simulink library "DAEMOT_Lib"  (R2019b)
settings: Solver=ode45  StartTime=0.0  StopTime=10.0  FixedStep=0.1  RelTol=1e-3
undefined symbols (not defined in the file or in its folder): Controller, CP, Ctrl, Ctrl_Fcn, Elec1, f, F2, Fluid, lag1, Mission, Moody, PropellerProp, rev_comms_sink
libraries: $bdroot x200, instrumentlib x21, simulink x5, dspsigops x2
(part 2 of 13)

== system DAEMOT_Lib/Electrical ==
  Air Vehicle : Subsystem  mask{rho=1.225, g=9.81, M=85, A=2*pi*(1/3)^2, d=.625, C_D=1.5/90, C_T=.07, C_tau=.01, eta=.95, theta=3.6, v_initial=30}
      mask prompts: rho "Air Density [kg/m^3]"; g "Gravity [m/s^2]"; M "Vehicle Mass [kg]"; A "Frontal Area [m^2]"; d "Prop Diameter"; C_D "Drag Coefficient [-]"; C_T "Thrust Coefficient [-]"; C_tau "Torque Coefficient [-]"; eta "Prop Efficiency [-]"; theta "Angle of attack [degrees]"; v_initial "Initial Vehicle Speed [m/s]"
      mask init:
      | % map = load('PropellerProp','PropellerProp');
      | % Prop = eval(['map.PropellerProp.' prop]);
      | % d = Prop.d;
      settings: CopyFcn=|
      | h      = get_param(gcb,'handle');   % Get block handle
      | blk    = gcb;
      | 
      | set_param(blk, 'LinkStatus', 'inactive')
      | clear h
      | clear blk
      mask DialogControl ParameterTabVar0 Prompt: Vehicle Parameters
      mask DialogControl ParameterTabVar012 Prompt: System
      mask Display:
      | image(imread('UAV.bmp'));
      | text(0.5,0.95,['{\bf UAV}'],'TexMode','on','horizontalAlignment', 'center')
      | text(0.5,0.075,['{\bf (\tau)  (end)}'],'TexMode','on','horizontalAlignment', 'center')
      | 
      | port_label('input',1,sprintf('Mechanical \nIn'))
      | 
      | % port_label('input',2,'\theta [rad]','interpreter','tex')
  Battery : Subsystem  AncestorBlock=DAEMOT_Lib_Copy/Dyn Electrical Comp/Battery  mask{C_c=62.7, C_s=4.5, R_cond=1.94, B_cap=21.33, Ns=3, Np=2, batt=57.6 Testbed 21.33 Ah, Ts_initial=25, Tc_initial=25, SOC_initial=.75, RC_initial=[0 0]}
      mask prompts: C_c "Lumped Cell Core Heat Capacity [J/K]"; C_s "Lumped Cell Surface Heat Capacity [J/K]"; R_cond "Conduction Resistance  [K/W]"; B_cap "Battery Capacity [Ah]"; Ns "Number of Cells (Series)"; Np "Number of Cells (Parallel)"; batt "Battery Type"; Ts_initial "Initial Battery Surface Temperature [C]"; Tc_initial "Initial Battery Core Temperature [C]"; SOC_initial "Initial State of Charge"; RC_initial "Initial RC Pair Voltage"
      mask init:
      | load('BattProp.mat');
      | 
      | if strcmp(batt,'3.3V LiFePO4 2.3 Ah')
      |     cell = BattProp.LiFePO_33V;
      |     t = 1;
      | end
      | 
      | if strcmp(batt,'3.3V LiFePO4 Graph 2.3 Ah')
      |     cell = BattProp.LiFePO_33V_G;
      |     t = 2;
      | end
      | 
      | if strcmp(batt,'4.2V LiPo 5.1 Ah')
      |     cell = BattProp.LiPo_42V;
      |     t = 1;
      | end
      | 
      | if strcmp(batt,'4.2V LiPo Graph 5.1 Ah')
      |     cell = BattProp.LiPo_42V_G;
      |     t = 2;
      | end
      | 
      | if strcmp(batt,'57.6 Testbed 21.33 Ah')
      |     cell = BattProp.Testbed4Pack;
      |     t = 1;
      | end
      | 
      | if strcmp(batt,'57.6 Testbed Graph 21.33 Ah')
      |     cell = BattProp.Testbed4Pack_G;
      |     t = 2;
      | end
      | 
      | 
      | % B_cap = B_cap*Np;
      | % C_c = C_c*Np*Ns;
      | % C_s = C_s*Np*Ns;
      | % R_cond = R_cond/(Np*Ns);
      settings: CopyFcn=|
      | h      = get_param(gcb,'handle');   % Get block handle
      | blk    = gcb;
      | 
      | set_param(blk, 'LinkStatus', 'inactive')
      | clear h
      | clear blk
      mask TypeOptions batt: 3.3V LiFePO4 2.3 Ah | 3.3V LiFePO4 Graph 2.3 Ah | 4.2V LiPo 5.1 Ah | 4.2V LiPo Graph 5.1 Ah | 57.6 Testbed 21.33 Ah | 57.6 Testbed Graph 21.33 Ah
      mask DialogControl ParameterTabVar0 Prompt: Module Parameters
      mask DialogControl ParameterTabVar01 Prompt: Initial Conditions
      mask DialogControl ParameterTabVar012 Prompt: System
      mask Display:
      | image(imread('battery.bmp'))
      | N = get_param(gcb,'Np');
      | M = get_param(gcb,'Ns');
      | 
      | text(0.5,0.95,[M '{\bfS}' N '{\bfP Battery}'],'TexMode','on','horizontalAlignment', 'center')
      | text(0.5,0.075,['{\bf (V)*}'],'TexMode','on','horizontalAlignment', 'center')
      | 
      | port_label('input',1,sprintf('Electrical \nIn'))
      | 
      | port_label('output',1,sprintf('Electrical \nOut'))
      | port_label('output',2,sprintf('Cooling \nOut'))
  Bus : Subsystem  mask{R=.1, L=.0001, C=1, Num_In=2, Num_Out=2, V_initial=.5, I_initial=0}
      mask prompts: R "Resistance [Ohm]"; L "Inductance [H]"; C "Capacitance [F]"; Num_In "Number of Inputs"; Num_Out "Number of Outputs"; V_initial "Initial Voltage [V]"; I_initial "Initial Current [A]"
      mask init:
      | h      = get_param(gcb,'handle');   % Get block handle
      | blk    = gcb;
      | hblock = get(h);     % Parse out handles structure
      | 
      | %%%%%%%%%%%%%%%%%%%%%%%%%%%%%% Clear Stuff %%%%%%%%%%%%%%%%%%%%%%%%%%%%%%%%
      | %delete any previous inports and bus selectors
      | for i = str2num(hblock.Num_In)+1:hblock.Ports(1)-2
      |     delete_block([blk,'/In',num2str(i)])
      |     delete_block([blk,'/gb',num2str(i)])
      |     delete_block([blk,'/vm',num2str(i)])
      |     delete_block([blk,'/term',num2str(i)])
      |     delete_block([blk,'/Sink',num2str(i)])
      |     delete_block([blk,'/vin',num2str(i)])
      |     
      |     delete_unconnected_lines(blk)
      | end
      | 
      | for i = str2num(hblock.Num_Out)+1:hblock.Ports(2)
      |     delete_block([blk,'/Out',num2str(i)])
      |     delete_block([blk,'/if',num2str(i)])
      |     delete_block([blk,'/io',num2str(i)])
      |     delete_block([blk,'/vo',num2str(i)])
      |     delete_block([blk,'/vot',num2str(i)])
      |     delete_block([blk,'/b',num2str(i)])
      |     delete_block([blk,'/Source',num2str(i)])
      |     delete_block([blk,'/ig',num2str(i)])
      |     delete_block([blk,'/ios',num2str(i)])
      |     
      |     delete_unconnected_lines(blk)
      | end
      | %%%%%%%%%%%%%%%%%%%%%%%%%%%%% Clear Stuff %%%%%%%%%%%%%%%%%%%%%%%%%%%%%%%%
      | 
      | %%%%%%%%%%%%%%%%%%%%%%%%%%%%%% Edit Mux inputs %%%%%%%%%%%%%%%%%%%%%%%%%%%%%%%%
      | set_param([blk,'/Mux_In_1'],'Inputs',hblock.Num_In)
      | set_param([blk,'/Mux_In_2'],'Inputs',hblock.Num_Out)
      | set_param([blk,'/Demux_Out_1'],'Outputs',hblock.Num_In)
      | set_param([blk,'/Demux_Out_2'],'Outputs',hblock.Num_Out)
      | set_param([blk,'/u_Out'],'Port',num2str(Num_In+2))
      | set_param([blk,'/u_In'],'Port',num2str(Num_In+1))
      | set_param([blk,'/Bus_Sink_1'],'Inputs',num2str(str2num(hblock.Num_Out)+1))
      | 
      | %%%%%%%%%%%%%%%%%%%%%%%%%%%%%% Edit Mux inputs %%%%%%%%%%%%%%%%%%%%%%%%%%%%%%%%
      | 
      | %%%%%%%%%%%%%%%%%%%%%%%%%%%%%% Create and Place Inputs %%%%%%%%%%%%%%%%%%%%%%%%%%%%%%%%
      | % generate inports, bus selectors, and route lines to each vector concat
      | for i = hblock.Ports(1)+1-2:str2num(hblock.Num_In)
      |     
      |     % add blocks (positioning notation [x i*s+y x+l i*s+h+y] x:(horiz. pos.), y:(vert. pos.), s:(spacing), l:(horiz. length), x:(vert. height)
      |     add_block('simulink/Ports & Subsystems/In1',   [blk,'/In',num2str(i)],    'Position',[355 i*80+425 355+30 i*80+13+425]);         % adding inport
      |     add_block([blk,'/gb1'],                        [blk,'/gb',num2str(i)],   'Position',[440 i*80+410 440+5 i*80+38+410]);         % adding inport
      |     add_block('simulink/Signal Routing/Goto',      [blk,'/vm',num2str(i)],    'Position',[500 i*80+450 500+80 i*80+14+450]);         % adding inport
      |     add_block('simulink/Sinks/Terminator',          [blk,'/term',num2str(i)],    'Position',[500 i*80+415 500+20 i*80+14+415]);         % adding inport
      |     add_block('DAEMOT_Lib/Support Functions/Sink',[blk,'/Sink',num2str(i)],'Position',[200 i*30+336 200+65 i*30+28+336]);         % adding inport
      |     add_block('simulink/Signal Routing/From',       [blk,'/vin',num2str(i)],     'Position',[-400 i*20+405 -400+80 i*20+18+405]);         % adding inport
      |     
      |     % set goto and from tags
      |     set_param([blk,'/vm',num2str(i)],'GotoTag',char(horzcat('V_in',num2str(i))))
      |     set_param([blk,'/vin',num2str(i)],'GotoTag',char(horzcat('V_in',num2str(i))))
      |     
      |     % set goto and from background colors
      | %    set_param([blk,'/gm',num2str(i)],'BackgroundColor','yellow')
      | %    set_param([blk,'/gt',num2str(i)],'BackgroundColor','yellow')
      | %    %set_param([blk,'/gp',num2str(i)],'BackgroundColor','yellow')
      | %    set_param([blk,'/min',num2str(i)],'BackgroundColor','yellow')
      | %    set_param([blk,'/tin',num2str(i)],'BackgroundColor','yellow')
      | %    set_param([blk,'/pout',num2str(i)],'BackgroundColor','cyan')
      |     
      |     % add lines
      |     add_line(blk,['In',num2str(i),'/1'], ['gb',num2str(i),'/1'],'AutoRouting','on')
      |     add_line(blk,['gb',num2str(i),'/2'],  ['vm',num2str(i),'/1'],'AutoRouting','on')
      |     add_line(blk,['gb',num2str(i),'/1'],  ['term',num2str(i),'/1'],'AutoRouting','on')
      |     add_line(blk,['Demux_Out_1/',num2str(i)],  ['Sink',num2str(i),'/1'],'AutoRouting','on')
      |     add_line(blk,['vin',num2str(i),'/1'],  ['Mux_In_1/',num2str(i)],'AutoRouting','on')
      | %     
      | end
      | %%%%%%%%%%%%%%%%%%%%%%%%%%%%%% Create and Place Inputs %%%%%%%%%%%%%%%%%%%%%%%%%%%%%%%%
      | 
      | %%%%%%%%%%%%%%%%%%%%%%%%%%%%%% Create and Place Outputs %%%%%%%%%%%%%%%%%%%%%%%%%%%%%%%%
      | % generate inports, bus selectors, and route lines to each vector concat
      | for i = hblock.Ports(2)+1:str2num(hblock.Num_Out)
      |     
      |     % add blocks
      |     add_block('simulink/Ports & Subsystems/Out1',   [blk,'/Out',num2str(i)],   'Position',[875 i*80+425 875+30 i*80+13+425]);         % adding inport
      |     add_block('simulink/Signal Routing/Bus Creator',[blk,'/b',num2str(i)],     'Position',[825 i*80+410 825+5 i*80+38+410]);         % adding inport
      |     add_block('simulink/Signal Routing/From',       [blk,'/io',num2str(i)],     'Position',[710 i*80+415 710+80 i*80+14+415]);         % adding inport
      |     add_block('simulink/Signal Routing/From',       [blk,'/vo',num2str(i)],     'Position',[710 i*80+435 710+80 i*80+14+435]);         % adding inport
      |     add_block('simulink/Signal Routing/Goto',       [blk,'/vot',num2str(i)],     'Position',[1250 i*20+50 1250+80 i*20+18+50]);         % adding inport
      |     add_block('simulink/Signal Routing/From',       [blk,'/if',num2str(i)],     'Position',[935 i*20+410 935+80 i*20+18+410]);         % adding inport
      |     add_block('DAEMOT_Lib/Support Functions/Source',[blk,'/Source',num2str(i)],'Position',[1400 i*30+420 1400+65 i*30+28+420]);         % adding inport
      |     add_block('simulink/Signal Routing/Goto',       [blk,'/ig',num2str(i)],     'Position',[1550 i*30+430 1550+80 i*30+14+430]);         % adding inport
      |     add_block('simulink/Signal Routing/From',       [blk,'/ios',num2str(i)],     'Position',[1770 i*16+405 1770+80 i*16+14+405]);         % adding inport
      |     
      |     % set goto and from tags
      |     set_param([blk,'/if',num2str(i)],'GotoTag',char(horzcat('I_out',num2str(i))))
      |     set_param([blk,'/io',num2str(i)],'GotoTag',char(horzcat('I_out',num2str(i))))
      |     set_param([blk,'/vo',num2str(i)],'GotoTag',char(horzcat('V_out',num2str(i))))
      |     set_param([blk,'/vot',num2str(i)],'GotoTag',char(horzcat('V_out',num2str(i))))
      |     set_param([blk,'/ig',num2str(i)],'GotoTag',char(horzcat('I_out',num2str(i))))
      |     set_param([blk,'/ios',num2str(i)],'GotoTag',char(horzcat('I_out',num2str(i))))
      |     set_param([blk,'/b',num2str(i)],'Inputs','2')
      |     
      | %     % set goto and from background colors
      | %     set_param([blk,'/t',num2str(i)],'BackgroundColor','cyan')
      | %     set_param([blk,'/m',num2str(i)],'BackgroundColor','cyan')
      | %     set_param([blk,'/p',num2str(i)],'BackgroundColor','cyan')
      | %     set_param([blk,'/g',num2str(i)],'BackgroundColor','cyan')
      | %     set_param([blk,'/mout',num2str(i)],'BackgroundColor','cyan')
      | %     %set_param([blk,'/tout',num2str(i)],'BackgroundColor','cyan')
      |     
      |     % add lines
      |     add_line(blk,['io',num2str(i),'/1'],['b',num2str(i),'/1'],'AutoRouting','on')
      |     p = get_param([blk,'/io',num2str(i)],'PortHandles');
      |     l = get_param(p.Outport,'Line');
      |     set_param(l,'Name','current')
      |     
      |     add_line(blk,['vo',num2str(i),'/1'],['b',num2str(i),'/2'],'AutoRouting','on')
      |     p = get_param([blk,'/vo',num2str(i)],'PortHandles');
      |     l = get_param(p.Outport,'Line');
      |     set_param(l,'Name','voltage')
      |         
      |     add_line(blk,['ios',num2str(i),'/1'],['Bus_Sink_1/',num2str(i+1)],'AutoRouting','on')
      |     p = get_param([blk,'/ios',num2str(i)],'PortHandles');
      |     l = get_param(p.Outport,'Line');
      |     set_param(l,'Name',['Current',num2str(i)])
      |      
      |     add_line(blk,['b',num2str(i),'/1'],['Out',num2str(i),'/1'],'AutoRouting','on')
      |     add_line(blk,['Source',num2str(i),'/1'],['ig',num2str(i),'/1'],'AutoRouting','on')
      |     add_line(blk,['if',num2str(i),'/1'],  ['Mux_In_2/',num2str(i)],'AutoRouting','on')
      |     add_line(blk,['Demux_Out_2/',num2str(i)],['vot',num2str(i),'/1'],'AutoRouting','on')
      |     
      | 
      | 
      | end
      | %%%%%%%%%%%%%%%%%%%%%%%%%%%%%% Create and Place Outputs %%%%%%%%%%%%%%%%%%%%%%%%%%%%%%%%
      | 
      | try
      |     set_param([blk,'/Selector1'],'InputPortWidth',num2str(hblock.Num_In))
      |     
      |     selector_str = '[1 ';
      |     for i = 2:str2num(hblock.Num_In)
      |         selector_str = [selector_str,num2str(i),' '];
      |     end
      |     selector_str = [selector_str,']'];
      |     set_param([blk,'/Selector1'],'IndexParamArray',{selector_str})%num2cell(1:hblock.Num_In))
      | catch
      |     selector_str = '[1 ';
      |     for i = 2:str2num(hblock.Num_In)
      |         selector_str = [selector_str,num2str(i),' '];
      |     end
      |     selector_str = [selector_str,']'];
      |     set_param([blk,'/Selector1'],'IndexParamArray',{selector_str})%num2cell(1:hblock.Num_In))
      |     
      |     set_param([blk,'/Selector1'],'InputPortWidth',num2str(hblock.Num_In))
      | end 
      |     
      | try
      |     set_param([blk,'/Selector2'],'InputPortWidth',num2str(hblock.Num_Out))
      |     
      |     selector_str = '[1 ';
      |     for i = 2:str2num(hblock.Num_Out)
      |         selector_str = [selector_str,num2str(i),' '];
      |     end
      |     selector_str = [selector_str,']'];
      |     set_param([blk,'/Selector2'],'IndexParamArray',{selector_str})%num2cell(1:hblock.Num_Out))
      | catch
      |     selector_str = '[1 ';
      |     for i = 2:str2num(hblock.Num_Out)
      |         selector_str = [selector_str,num2str(i),' '];
      |     end
      |     selector_str = [selector_str,']'];
      |     set_param([blk,'/Selector2'],'IndexParamArray',{selector_str})%num2cell(1:hblock.Num_Out))
      |     
      |     set_param([blk,'/Selector2'],'InputPortWidth',num2str(hblock.Num_Out))
      | end 
      | 
      |     clear h blk hblock
      settings: CopyFcn=|
      | h      = get_param(gcb,'handle');   % Get block handle
      | blk    = gcb;
      | 
      | set_param(blk, 'LinkStatus', 'inactive')
      | clear h
      | clear blk
      mask DialogControl ParameterTabVar0 Prompt: Bus Parameters
      mask DialogControl ParameterTabVar01 Prompt: System
      mask Display:
      | text(0.5,0.95,['{\bf Bus}'],'TexMode','on','horizontalAlignment', 'center')
      | text(0.5,0.075,['{\bf ----(V)}'],'TexMode','on','horizontalAlignment', 'center')
      | 
      | In = get_param(gcb,'Num_In');
      | Out = get_param(gcb,'Num_Out');
      | 
      | for i = 1:str2num(In)
      |     port_label('input',i,sprintf(['Electrical \nIn ',num2str(i)]))
      | end
      | port_label('input',str2num(In)+1,'u In')
      | port_label('input',str2num(In)+2,'u Out')
      | 
      | for i = 1:str2num(Out)
      |     port_label('output',i,sprintf(['Electrical \nOut ',num2str(i)]))
      | end
  Capacitor : Subsystem  mask{C=1, V_initial=0}
      mask prompts: C "Capacitance [F]"; V_initial "Initial Ouput Voltage [V]"
      mask init:
      | % if strcmp(Gn_check,'off')
      | %     %is not ground node
      | %     Gn = 0;
      | %     %V_initial = V_initial_temp;
      | % else
      | %     %is ground node
      | %     Gn = 1;
      | %     %V_initial = 0;
      | % end
      mask DialogControl ParameterTabVar0 Prompt: Capacitor Parameters
      mask DialogControl ParameterTabVar01 Prompt: System
      mask Display:
      | image(imread('capacitor.bmp'));
      | text(0.5,0.95,['{\bf Capacitor}'],'TexMode','on','horizontalAlignment', 'center')
      | text(0.5,0.075,['{\bf (V)}'],'TexMode','on','horizontalAlignment', 'center')
      | 
      | port_label('input',1,sprintf('Electrical \nIn'))
      | %port_label('input',2,'Capacitance')
      | port_label('output',1,sprintf('Electrical \nOut'))
  Converter : Subsystem  mask{V_D=.01, R_D=.01, R_s=.01, R_L=.01, dir=<===, Cp=60, T_initial=25}
      mask prompts: V_D "Diode Voltage Difference [V]"; R_D "Diode Resistance [Ohm]"; R_s "Switch Resistance [Ohm]"; R_L "Copper Loss [Ohm]"; dir "Conversion Direction (Boost)"; Cp "Heat Capacity [J/K]"; T_initial "Initial Temperature [C]"
      mask TypeOptions dir: ===> | <===
      mask DialogControl ParameterTabVar0 Prompt: Model Parameters
      mask DialogControl ParameterTabVar01 Prompt: Cooling
      mask DialogControl ParameterTabVar012 Prompt: System
      mask Display:
      | image(imread('converter.bmp'));
      | text(0.5,0.95,['{\bf BuckBoost Converter}'],'TexMode','on','horizontalAlignment', 'center')
      | text(0.5,0.075,['{\bf ----(V)}'],'TexMode','on','horizontalAlignment', 'center')
      | dir = get_param(gcb,'dir');
      | 
      | switch dir
      |     case '===>'
      |         text(0.5,0.85,['{\bf Boost[1] ===>}'],'TexMode','on','horizontalAlignment', 'center')
      |         text(0.5,0.75,['{\bf Buck[0] <===}'],'TexMode','on','horizontalAlignment', 'center')
      |     case '<==='
      |         text(0.5,0.85,['{\bf Boost[1] <===}'],'TexMode','on','horizontalAlignment', 'center')
      |         text(0.5,0.75,['{\bf Buck[0] ===>}'],'TexMode','on','horizontalAlignment', 'center')
      | end
      | 
      | 
      | 
      | port_label('input',1,sprintf('Electrical \nIn'))
      | port_label('input',2,sprintf('Duty \nCycle'))
      | port_label('input',3,sprintf('Operating \nMode'))
      | port_label('output',1,sprintf('Electrical \nOut'))
      | port_label('output',2,sprintf('Cooling \nOut'))
  Cooling Sink : Subsystem  Commented=on  mask(Effort Sink (Torque)){M_ext=on, M=0, T_ext=on, T=0, P_ext=on, P=0}
      mask prompts: M_ext "Mass flow rate time varying?"; M "Mass flow rate (kg/s)"; T_ext "Temperature time varying?"; T "Temperature (C)"; P_ext "Pressure time varying?"; P "Pressure (kPa)"
      mask help: Used to create a effot sink.
      mask Callback M_ext:
      | en = get_param(gcb,'MaskVisibilities');
      | h      = get_param(gcb,'handle');   % Get block handle
      | blk    = gcb;
      | hblock = get(h);     % Parse out handles structure
      | 
      | switch get_param(gcb,'M_ext')
      |     case 'on'
      |         en{2} = 'off';
      |         %add_block('simulink/Ports & Subsystems/In1',   [blk,'/In1'],'Position',[130    -7   160     7]);         % adding inport
      | 
      |     case 'off'
      |         en{2} = 'on';
      |         %delete_block([blk,'/In1'])
      | 
      | end
      | set_param(gcb,'MaskVisibilities',en);
      mask Callback T_ext:
      | en = get_param(gcb,'MaskVisibilities');
      | 
      | switch get_param(gcb,'T_ext')
      |     case 'on'
      |         en{4} = 'off';
      |     case 'off'
      |         en{4} = 'on';
      | end
      | set_param(gcb,'MaskVisibilities',en);
      mask Callback P_ext:
      | en = get_param(gcb,'MaskVisibilities');
      | 
      | switch get_param(gcb,'P_ext')
      |     case 'on'
      |         en{6} = 'off';
      |     case 'off'
      |         en{6} = 'on';
      | end
      | set_param(gcb,'MaskVisibilities',en);
      mask Display:
      | text(0.5,0.95,['{\bf Flow Sink}'],'TexMode','on','horizontalAlignment', 'center')
      | text(0.5,0.1,['{(----)(end)}'],'TexMode','on','horizontalAlignment', 'center')
      | 
      | port_label('input',1,'Sink')
      | port_label('input',2,'Sink Heat Flow [kW]')
  Cooling Source : Subsystem  Commented=on  mask(Cooling Source){M_ext=on, M=0, T_ext=on, T=0, P_ext=on, P=0}
      mask prompts: M_ext "Mass flow rate time varying?"; M "Mass flow rate (kg/s)"; T_ext "Temperature time varying?"; T "Temperature (C)"; P_ext "Pressure time varying?"; P "Pressure (kPa)"
      mask help: Used to create an cooling source.
      mask Callback M_ext:
      | en = get_param(gcb,'MaskVisibilities');
      | h      = get_param(gcb,'handle');   % Get block handle
      | blk    = gcb;
      | hblock = get(h);     % Parse out handles structure
      | 
      | switch get_param(gcb,'M_ext')
      |     case 'on'
      |         en{2} = 'off';
      |         %add_block('simulink/Ports & Subsystems/In1',   [blk,'/In1'],'Position',[130    -7   160     7]);         % adding inport
      | 
      |     case 'off'
      |         en{2} = 'on';
      |         %delete_block([blk,'/In1'])
      | 
      | end
      | set_param(gcb,'MaskVisibilities',en);
      mask Callback T_ext:
      | en = get_param(gcb,'MaskVisibilities');
      | 
      | switch get_param(gcb,'T_ext')
      |     case 'on'
      |         en{4} = 'off';
      |     case 'off'
      |         en{4} = 'on';
      | end
      | set_param(gcb,'MaskVisibilities',en);
      mask Callback P_ext:
      | en = get_param(gcb,'MaskVisibilities');
      | 
      | switch get_param(gcb,'P_ext')
      |     case 'on'
      |         en{6} = 'off';
      |     case 'off'
      |         en{6} = 'on';
      | end
      | set_param(gcb,'MaskVisibilities',en);
      mask Display:
      | text(0.5,0.95,['{\bf Effort Source}'],'TexMode','on','horizontalAlignment', 'center')
      | text(0.5,0.1,['{(start)(----)}'],'TexMode','on','horizontalAlignment', 'center')
      | 
      | port_label('input',1,sprintf('Source Heat \nFlow [kW]')  )
      | 
      | port_label('output',1,'Source')
  Current Sink : Subsystem  Commented=on  mask(Flow Sink (Current)){M_ext=on, M=0, T_ext=on, T=0, P_ext=on, P=0}
      mask prompts: M_ext "Mass flow rate time varying?"; M "Mass flow rate (kg/s)"; T_ext "Temperature time varying?"; T "Temperature (C)"; P_ext "Pressure time varying?"; P "Pressure (kPa)"
      mask help: Used to create a flow sink.
      mask Callback M_ext:
      | en = get_param(gcb,'MaskVisibilities');
      | h      = get_param(gcb,'handle');   % Get block handle
      | blk    = gcb;
      | hblock = get(h);     % Parse out handles structure
      | 
      | switch get_param(gcb,'M_ext')
      |     case 'on'
      |         en{2} = 'off';
      |         %add_block('simulink/Ports & Subsystems/In1',   [blk,'/In1'],'Position',[130    -7   160     7]);         % adding inport
      | 
      |     case 'off'
      |         en{2} = 'on';
      |         %delete_block([blk,'/In1'])
      | 
      | end
      | set_param(gcb,'MaskVisibilities',en);
      mask Callback T_ext:
      | en = get_param(gcb,'MaskVisibilities');
      | 
      | switch get_param(gcb,'T_ext')
      |     case 'on'
      |         en{4} = 'off';
      |     case 'off'
      |         en{4} = 'on';
      | end
      | set_param(gcb,'MaskVisibilities',en);
      mask Callback P_ext:
      | en = get_param(gcb,'MaskVisibilities');
      | 
      | switch get_param(gcb,'P_ext')
      |     case 'on'
      |         en{6} = 'off';
      |     case 'off'
      |         en{6} = 'on';
      | end
      | set_param(gcb,'MaskVisibilities',en);
      mask Display:
      | text(0.5,0.95,['{\bf Flow Sink}'],'TexMode','on','horizontalAlignment', 'center')
      | text(0.5,0.1,['{(----) (end)}'],'TexMode','on','horizontalAlignment', 'center')
      | 
      | port_label('input',1,'Sink')
      | port_label('input',2,'Sink Current [A]')
  Current Source : Subsystem  Commented=on  mask(Current Source){M_ext=on, M=0, T_ext=on, T=0, P_ext=on, P=0}
      mask prompts: M_ext "Mass flow rate time varying?"; M "Mass flow rate (kg/s)"; T_ext "Temperature time varying?"; T "Temperature (C)"; P_ext "Pressure time varying?"; P "Pressure (kPa)"
      mask help: Used to create an flow source.
      mask Callback M_ext:
      | en = get_param(gcb,'MaskVisibilities');
      | h      = get_param(gcb,'handle');   % Get block handle
      | blk    = gcb;
      | hblock = get(h);     % Parse out handles structure
      | 
      | switch get_param(gcb,'M_ext')
      |     case 'on'
      |         en{2} = 'off';
      |         %add_block('simulink/Ports & Subsystems/In1',   [blk,'/In1'],'Position',[130    -7   160     7]);         % adding inport
      | 
      |     case 'off'
      |         en{2} = 'on';
      |         %delete_block([blk,'/In1'])
      | 
      | end
      | set_param(gcb,'MaskVisibilities',en);
      mask Callback T_ext:
      | en = get_param(gcb,'MaskVisibilities');
      | 
      | switch get_param(gcb,'T_ext')
      |     case 'on'
      |         en{4} = 'off';
      |     case 'off'
      |         en{4} = 'on';
      | end
      | set_param(gcb,'MaskVisibilities',en);
      mask Callback P_ext:
      | en = get_param(gcb,'MaskVisibilities');
      | 
      | switch get_param(gcb,'P_ext')
      |     case 'on'
      |         en{6} = 'off';
      |     case 'off'
      |         en{6} = 'on';
      | end
      | set_param(gcb,'MaskVisibilities',en);
      mask Display:
      | text(0.5,0.95,['{\bf Flow Source}'],'TexMode','on','horizontalAlignment', 'center')
      | text(0.5,0.1,['{(start) (----)}'],'TexMode','on','horizontalAlignment', 'center')
      | 
      | %port_label('input',1,'Source Current [A]')
      | port_label('input',1,sprintf('Source \nCurrent [A]'))
      | 
      | port_label('output',1,'Source')
  ESC : Subsystem  mask{esc=NoDyno}
      mask prompts: esc "ESC Background Loss Map (filename)"
      mask init:
      | map = load('EscProp','EscProp');
      | Esc = eval(['map.EscProp.' esc]);
      settings: CopyFcn=|
      | h      = get_param(gcb,'handle');   % Get block handle
      | blk    = gcb;
      | 
      | set_param(blk, 'LinkStatus', 'inactive')
      | clear h
      | clear blk
      mask TypeOptions esc: All | NoDyno
      mask DialogControl ParameterTabVar0 Prompt: Vehicle Parameters
      mask DialogControl ParameterTabVar012 Prompt: System
      mask Display:
      | image(imread('ESC.bmp'));
      | text(0.5,0.95,['{\bf ESC Background}'],'TexMode','on','horizontalAlignment', 'center')
      | text(0.5,0.85,['{\bf Loss}'],'TexMode','on','horizontalAlignment', 'center')
      | text(0.5,0.075,['{\bf ---- (end)}'],'TexMode','on','horizontalAlignment', 'center')
      | 
      | port_label('input',1,sprintf('Electrical \nIn'))
      | % port_label('input',2,sprintf('\\lambda %g\t',10))
      | % port_label('input',2,'\theta [rad]','interpreter','tex')
  Effort Sink : Subsystem  Commented=on  mask(Effort Sink (Torque)){Stype=Voltage Sink, const=on, value=0}
      mask prompts: Stype "Sink Type"; const "Constant Value?"; value "Voltage [V]"
      mask help: Used to create a effot sink.
      mask init:
      | h      = get_param(gcb,'handle');   % Get block handle
      | blk    = gcb;
      | hblock = get(h);     % Parse out handles structure
      | 
      | if const == 1;
      |     try delete_block([blk,'/In2'])
      |         delete_unconnected_lines(blk);
      |         add_block('simulink/Sources/Constant',   [blk,'/val'], 'Position', [200,218,230,232]);
      |         add_line(blk,'val/1','Sink1/1','AutoRouting','on');
      |         set_param([blk,'/val'],'Value','value');
      |     end
      |      
      | %     delete_unconnected_lines(blk)
      | else
      |     try delete_block([blk,'/val'])
      |         delete_unconnected_lines(blk);
      |         add_block('simulink/Ports & Subsystems/In1',   [blk,'/In2'], 'Position', [200,218,230,232]);
      |         add_line(blk,'In2/1','Sink1/1','AutoRouting','on');
      |     end
      | end
      | 
      | clear h blk hblock
      settings: CopyFcn=|
      | h      = get_param(gcb,'handle');   % Get block handle
      | blk    = gcb;
      | 
      | set_param(blk, 'LinkStatus', 'inactive')
      | clear h
      | clear blk
      mask TypeOptions Stype: Voltage Sink | Current Sink | Angular Speed Sink | Torque Sink | Temperature Sink | Heat Flow Sink
      mask Callback Stype:
      | mp = get_param(gcb,'MaskPrompts');
      | h      = get_param(gcb,'handle');   % Get block handle
      | blk    = gcb;
      | hblock = get(h);     % Parse out handles structure
      | 
      | switch get_param(gcb,'Stype')
      |     case 'Voltage Sink'
      |         mp{3} = 'Voltage [V]';
      |     case 'Current Sink'
      |         mp{3} = 'Current [A]';
      |     case 'Angular Speed Sink'
      |         mp{3} = 'Speed [rad/s]';
      |     case 'Torque Sink'
      |         mp{3} = 'Torque [Nm]';
      |     case 'Temperature Sink'
      |         mp{3} = 'Temperature [C]';
      |     case 'Heat Flow Sink'
      |         mp{3} = 'Heat Flow [kW]';
      | end
      | set_param(gcb,'MaskPrompts',mp);
      mask Callback const:
      | en = get_param(gcb,'MaskVisibilities');
      | h      = get_param(gcb,'handle');   % Get block handle
      | blk    = gcb;
      | hblock = get(h);     % Parse out handles structure
      | 
      | switch get_param(gcb,'const')
      |     case 'on'
      |         en{3} = 'on';
      | %         delete_block([blk,'/In1'])
      | 
      |     case 'off'
      |         en{3} = 'off';
      | %         add_block('simulink/Ports & Subsystems/In1',   [blk,'/In1'],'Position',[130    -7   160     7]);         % adding inport
      | 
      | end
      | set_param(gcb,'MaskVisibilities',en);
      | 
      | % hblock.MaskPrompts{3} = 'hello';
      mask Display:
      | text(0.45,0.90,['{\bf',get_param(gcb,'Stype'),'}'],'TexMode','on','horizontalAlignment', 'center')
      | % text(0.5,0.1,['{(T)(end)}'],'TexMode','on','horizontalAlignment', 'center')
      | 
      | type = get_param(gcb,'Stype');
      | switch type
      |         case 'Voltage Sink'
      |             nm = 'Voltage [V]';
      |             id = '(V)';
      |             un = 'V';
      |         case 'Current Sink'
      |             nm = 'Current [A]';
      |             id = '(----)';
      |             un = 'A';
      |         case 'Angular Speed Sink'
      |             nm = 'Speed [rad/s]';
      |             id = '(----)';
      |             un = 'rad/s';
      |         case 'Torque Sink'
      |             nm = 'Torque [Nm]';
      |             id = '(\tau)';
      |             un = 'Nm';
      |         case 'Temperature Sink'
      |             nm = 'Temperature [C]';
      |             id = '(T)';
      |             un = 'C';
      |         case 'Heat Flow Sink'
      |             nm = 'Heat Flow [kW]';
      |             id = '(----)';
      |             un = 'kW';
      | end
      | 
      | if strcmp(get_param(gcb,'const'),'on')
      |     text(0.75,0.500,['{\bf',get_param(gcb,'Value'),un,'}'],'TexMode','on','horizontalAlignment', 'center')
      | else
      |     port_label('input',2,sprintf(['Sink ',nm]));
      | end
      | 
      | 
      | port_label('input',1,'Sink');
      | text(0.5,0.175,['{',id,' (end)}'],'TexMode','on','horizontalAlignment', 'center');
  Effort Source : Subsystem  Commented=on  mask(Effort Source (Voltage)){Stype=Voltage Source, const=on, value=0}
      mask prompts: Stype "Source Type"; const "Constant Value?"; value "Voltage [V]"
      mask help: Used to create an effort source.
      mask init:
      | h      = get_param(gcb,'handle');   % Get block handle
      | blk    = gcb;
      | hblock = get(h);     % Parse out handles structure
      | 
      | switch Stype
      |     case 1
      |         up = 'current';
      |         dw = 'voltage';
      |     case 2
      |         dw = 'current';
      |         up = 'voltage';
      |     case 3
      |         up = 'torque';
      |         dw = 'aspeed';
      |     case 4
      |         dw = 'torque';
      |         up = 'aspeed';
      |     case 5
      |         up = 'Q_kW';
      |         dw = 'Temp';
      |     case 6
      |         dw = 'Q_kW';
      |         up = 'Temp';
      | end
      | 
      | if const == 1;
      |     try delete_block([blk,'/In1'])
      |         delete_unconnected_lines(blk);
      |         add_block('simulink/Sources/Constant',   [blk,'/val'], 'Position', [200,198,230,212]);
      |         add_line(blk,'val/1','b1/2','AutoRouting','on');
      |         set_param([blk,'/val'],'Value','value');
      | 
      |         p = get_param([blk,'/Constant'],'PortHandles');
      |         l = get_param(p.Outport,'Line');
      |         set_param(l,'Name',up);
      |         
      |         p = get_param([blk,'/val'],'PortHandles');
      |         l = get_param(p.Outport,'Line');
      |         set_param(l,'Name',dw);
      |     end
      |     p = get_param([blk,'/Constant'],'PortHandles');
      |     l = get_param(p.Outport,'Line');
      |     if strcmp(get_param(l,'name'),up)
      |     else
      |         set_param(l,'Name',up);
      |         
      |         p = get_param([blk,'/val'],'PortHandles');
      |         l = get_param(p.Outport,'Line');
      |         set_param(l,'Name',dw);
      |     end
      |      
      | %     delete_unconnected_lines(blk)
      | else
      |     try delete_block([blk,'/val'])
      |         delete_unconnected_lines(blk);
      |         add_block('simulink/Ports & Subsystems/In1',   [blk,'/In1'], 'Position', [200,198,230,212]);
      |         add_line(blk,'In1/1','b1/2','AutoRouting','on');
      |         
      |         p = get_param([blk,'/Constant'],'PortHandles');
      |         l = get_param(p.Outport,'Line');
      |         set_param(l,'Name',up);
      | 
      |         p = get_param([blk,'/In1'],'PortHandles');
      |         l = get_param(p.Outport,'Line');
      |         set_param(l,'Name',dw);
      |     end
      |     p = get_param([blk,'/Constant'],'PortHandles');
      |     l = get_param(p.Outport,'Line');
      |     if strcmp(get_param(l,'name'),up)
      |     else
      |         set_param(l,'Name',up);
      |         
      |         p = get_param([blk,'/In1'],'PortHandles');
      |         l = get_param(p.Outport,'Line');
      |         set_param(l,'Name',dw);
      |     end
      | end
      | 
      | clear h blk hblock
      settings: CopyFcn=|
      | h      = get_param(gcb,'handle');   % Get block handle
      | blk    = gcb;
      | 
      | set_param(blk, 'LinkStatus', 'inactive')
      | clear h
      | clear blk
      mask TypeOptions Stype: Voltage Source | Current Source | Angular Speed Source | Torque Source | Temperature Source | Heat Flow Source
      mask Callback Stype:
      | mp = get_param(gcb,'MaskPrompts');
      | h      = get_param(gcb,'handle');   % Get block handle
      | blk    = gcb;
      | hblock = get(h);     % Parse out handles structure
      | 
      | switch get_param(gcb,'Stype')
      |     case 'Voltage Source'
      |         mp{3} = 'Voltage [V]';
      |     case 'Current Source'
      |         mp{3} = 'Current [A]';
      |     case 'Angular Speed Source'
      |         mp{3} = 'Speed [rad/s]';
      |     case 'Torque Source'
      |         mp{3} = 'Torque [Nm]';
      |     case 'Temperature Source'
      |         mp{3} = 'Temperature [C]';
      |     case 'Heat Flow Source'
      |         mp{3} = 'Heat Flow [kW]';
      | end
      | set_param(gcb,'MaskPrompts',mp);
      mask Callback const:
      | en = get_param(gcb,'MaskVisibilities');
      | h      = get_param(gcb,'handle');   % Get block handle
      | blk    = gcb;
      | hblock = get(h);     % Parse out handles structure
      | 
      | switch get_param(gcb,'const')
      |     case 'on'
      |         en{3} = 'on';
      | %         delete_block([blk,'/In1'])
      | 
      |     case 'off'
      |         en{3} = 'off';
      | %         add_block('simulink/Ports & Subsystems/In1',   [blk,'/In1'],'Position',[130    -7   160     7]);         % adding inport
      | 
      | end
      | set_param(gcb,'MaskVisibilities',en);
      | 
      | % hblock.MaskPrompts{3} = 'hello';
      mask Display:
      | text(0.45,0.900,['{\bf',get_param(gcb,'Stype'),'}'],'TexMode','on','horizontalAlignment', 'center')
      | 
      | type = get_param(gcb,'Stype');
      | switch type
      |         case 'Voltage Source'
      |             nm = 'Voltage [V]';
      |             id = '(V)*';
      |             un = 'V';
      |         case 'Current Source'
      |             nm = 'Current [A]';
      |             id = '(----)';
      |             un = 'A';
      |         case 'Angular Speed Source'
      |             nm = 'Speed [rad/s]';
      |             id = '(----)';
      |             un = 'rad/s';
      |         case 'Torque Source'
      |             nm = 'Torque [Nm]';
      |             id = '(\tau)*';
      |             un = 'Nm';
      |         case 'Temperature Source'
      |             nm = 'Temperature [C]';
      |             id = '(T)';
      |             un = 'C';
      |         case 'Heat Flow Source'
      |             nm = 'Heat Flow [kW]';
      |             id = '(----)';
      |             un = 'kW';
      | end
      | 
      | if strcmp(get_param(gcb,'const'),'on')
      |     text(0.25,0.500,['{\bf',get_param(gcb,'Value'),un,'}'],'TexMode','on','horizontalAlignment', 'center')
      | else
      |     port_label('input',1,sprintf(['Source \n',nm]))
      | end
      | port_label('output',1,'Source')
      | text(0.5,0.175,['{(start) ',id,'}'],'TexMode','on','horizontalAlignment', 'center')
  Engine : Subsystem  mask{G=-1, I_coeffs=[0,63.288903716034200,0], B_coeffs=[-0.015150028280914,1.757501363754273], S_coeffs=[0.197172947336021,0.088505107520121,1.502179108800752e+03,0.246955231644008,-31.725066916739816,-20.969196076216960], tau=.5, I_initial=0}
      mask prompts: G "Current Gain"; I_coeffs "Current Coefficients"; B_coeffs "Current Bound Coefficients"; S_coeffs "SFC Coefficients"; tau "Time Constant [s]"; I_initial "Initial Current"
      mask init:
      | % SFC_max = max(2);
      | % u_min = min(1);
      | % SFC_min = min(2);
      | % 
      | % a = -(SFC_min-SFC_max)/(u_min^2);
      | % b = -2*a*u_min;
      | % c = SFC_max;
      | 
      | S = [S_coeffs(1)   S_coeffs(4)/2 S_coeffs(5)/2; ...
      |      S_coeffs(4)/2 S_coeffs(2)   S_coeffs(6)/2; ...
      |      S_coeffs(5)/2 S_coeffs(6)/2 S_coeffs(3)];
      mask DialogControl ParameterTabVar0 Prompt: Engine Parameters
      mask DialogControl ParameterTabVar012 Prompt: System
      mask Display:
      | image(imread('generator.bmp'));
      | text(0.5,0.95,['{\bf Engine}'],'TexMode','on','horizontalAlignment', 'center')
      | text(0.5,0.075,['{\bf (----) (end)}'],'TexMode','on','horizontalAlignment', 'center')
      | 
      | port_label('input',1,sprintf('Electrical \nIn'))
      | port_label('input',2,sprintf('Throttle \n[%%]'))
  Gearbox : Subsystem  Commented=on  AncestorBlock=DAEMOT_Lib_Copy/Dyn Electrical Comp/Gearbox  mask{R=5, dir=1}
      mask prompts: R "Gear Ratio"; dir "Type"
      mask init:
      | h      = get_param(gcb,'handle');   % Get block handle
      | blk    = gcb;
      | hblock = get(h);     % Parse out handles structure
      | 
      | 
      | if dir == 1
      |     set_param([blk,'/i1'],'GotoTag',char(horzcat('term')));
      |     set_param([blk,'/i2'],'GotoTag',char(horzcat('var_in')));
      |     set_param([blk,'/O1'],'GotoTag',char(horzcat('in_down')));
      |     set_param([blk,'/O2'],'GotoTag',char(horzcat('var_out')));
      |     
      |     set_param([blk,'/o1'],'GotoTag',char(horzcat('out_up')));
      |     p = get_param([blk,'/o1'],'PortHandles');
      |     l = get_param(p.Outport,'Line');
      |     set_param(l,'Name','Input Speed [rad_s]')
      |     
      |     set_param([blk,'/o2'],'GotoTag',char(horzcat('var_out')));
      |     p = get_param([blk,'/o2'],'PortHandles');
      |     l = get_param(p.Outport,'Line');
      |     set_param(l,'Name','Output Torque [Nm]')
      | else
      |     set_param([blk,'/i1'],'GotoTag',char(horzcat('var_in')));
      |     set_param([blk,'/i2'],'GotoTag',char(horzcat('term')));
      |     set_param([blk,'/O1'],'GotoTag',char(horzcat('var_out')));
      |     set_param([blk,'/O2'],'GotoTag',char(horzcat('in_down')));
      |     
      |     set_param([blk,'/o1'],'GotoTag',char(horzcat('var_out')));
      |     p = get_param([blk,'/o1'],'PortHandles');
      |     l = get_param(p.Outport,'Line');
      |     set_param(l,'Name','Output Speed [rad_s]')
      |     
      |     set_param([blk,'/o2'],'GotoTag',char(horzcat('out_up')));
      |     p = get_param([blk,'/o2'],'PortHandles');
      |     l = get_param(p.Outport,'Line');
      |     set_param(l,'Name','Input Torque [Nm]')
      | end
      settings: CopyFcn=|
      | h      = get_param(gcb,'handle');   % Get block handle
      | blk    = gcb;
      | 
      | set_param(blk, 'LinkStatus', 'inactive')
      | clear h
      | clear blk
      mask TypeOptions dir: 1 | 2
      mask DialogControl ParameterTabVar0 Prompt: Gearbox Parameters
      mask DialogControl ParameterTabVar012 Prompt: System
      mask Display:
      | image(imread('Gearbox.bmp'));
      | text(0.5,0.95,['{\bf Gearbox}'],'TexMode','on','horizontalAlignment', 'center')
      | dir = get_param(gcb,'dir');
      | 
      | switch dir
      |     case '1'
      |         text(0.5,0.075,['{\bf ----(\tau)}'],'TexMode','on','horizontalAlignment', 'center')
      |     case '2'
      |         text(0.5,0.075,['{\bf (\tau)----}'],'TexMode','on','horizontalAlignment', 'center')
      | end
      | 
      | 
      | 
      | port_label('input',1,sprintf('Mech. \nIn'))
      | port_label('output',1,sprintf('Mech. \nOut'))
  Generator : Subsystem  Commented=on  mask{G=2.25}
      mask prompts: G "Current Gain"
      mask init:
      | load('Eng3W.mat')
      | 
      | cI = Eng3W.cI;
      | cSFC = Eng3W.cSFC;
      | mu_V = Eng3W.mu_V;
      | std_V = Eng3W.std_V;
      | mu_u = Eng3W.mu_u;
      | std_u = Eng3W.std_u;
      mask DialogControl ParameterTabVar0 Prompt: Generator Parameters
      mask DialogControl ParameterTabVar012 Prompt: System
      mask Display:
      | image(imread('generator.bmp'));
      | text(0.5,0.95,['{\bf Generator}'],'TexMode','on','horizontalAlignment', 'center')
      | text(0.5,0.075,['{\bf (--)}'],'TexMode','on','horizontalAlignment', 'center')
      | 
      | port_label('input',1,sprintf('Electrical \nIn'))
      | port_label('input',2,sprintf('Throttle \n[%%]'))
  Ground Vehicle : Subsystem  mask{R=.3, Af=2, rho_air=1.2, Cd=.26}
      mask prompts: R "Wheel Radius [m]"; Af "Frontal Area [m^2]"; rho_air "Air Density [kg/m^3]"; Cd "Drag Coefficient [-]"
      mask init:
      | % if strcmp(Gn_check,'off')
      | %     %is not ground node
      | %     Gn = 0;
      | %     %V_initial = V_initial_temp;
      | % else
      | %     %is ground node
      | %     Gn = 1;
      | %     %V_initial = 0;
      | % end
      mask DialogControl ParameterTabVar0 Prompt: Capacitor Parameters
      mask DialogControl ParameterTabVar01 Prompt: System
      mask Display:
      | image(imread('ground.bmp'));
      | text(0.5,0.95,['{\bf Ground Vehicle}'],'TexMode','on','horizontalAlignment', 'center')
      | text(0.5,0.075,['{\bf (T)  (end)}'],'TexMode','on','horizontalAlignment', 'center')
      | 
      | port_label('input',1,sprintf('Mechanical \nIn'))
      | port_label('input',2,sprintf('Brake \nTorque [Nm]'))
  Inductor : Subsystem  mask{L=1, I_initial=0}
      mask prompts: L "Inductance [H]"; I_initial "Initial Current [A]"
      mask init:
      | % if strcmp(Gn_check,'off')
      | %     %is not ground node
      | %     Gn = 0;
      | %     %V_initial = V_initial_temp;
      | % else
      | %     %is ground node
      | %     Gn = 1;
      | %     %V_initial = 0;
      | % end
      mask DialogControl ParameterTabVar0 Prompt: Capacitor Parameters
      mask DialogControl ParameterTabVar01 Prompt: System
      mask Display:
      | image(imread('inductor.bmp'));
      | text(0.5,0.95,['{\bf Inductor}'],'TexMode','on','horizontalAlignment', 'center')
      | text(0.5,0.075,['{\bf ----}'],'TexMode','on','horizontalAlignment', 'center')
      | 
      | port_label('input',1,sprintf('Electrical \nIn'))
      | %port_label('input',2,'Inductance')
      | port_label('output',1,sprintf('Electrical \nOut'))
  Inverter : Subsystem  mask{R_m=.0808, Cp=10000, T_initial=25}
      mask prompts: R_m "Modulated Loss [Ohm]"; Cp "Heat Capacity [J/K]"; T_initial "Initial Temperature [C]"
      settings: CopyFcn=|
      | h      = get_param(gcb,'handle');   % Get block handle
      | blk    = gcb;
      | 
      | set_param(blk, 'LinkStatus', 'inactive')
      | clear h
      | clear blk
      mask DialogControl DescTextVar Prompt: This is a wye configured inverter.
      mask DialogControl ParameterTabVar0 Prompt: Inverter Parameters
      mask DialogControl ParameterTabVar01 Prompt: Cooling
      mask DialogControl ParameterTabVar012 Prompt: System
      mask Display:
      | image(imread('inverter.bmp'));
      | text(0.5,0.95,['{\bf Inverter}'],'TexMode','on','horizontalAlignment', 'center')
      | text(0.5,0.075,['{\bf ----(V)}'],'TexMode','on','horizontalAlignment', 'center')
      | 
      | 
      | % switch dir
      | %     case '===>'
      | %         text(0.5,0.85,['{\bf Boost[1] ===>}'],'TexMode','on','horizontalAlignment', 'center')
      | %         text(0.5,0.75,['{\bf Buck[0] <===}'],'TexMode','on','horizontalAlignment', 'center')
      | %     case '<==='
      | %         text(0.5,0.85,['{\bf Boost[1] <===}'],'TexMode','on','horizontalAlignment', 'center')
      | %         text(0.5,0.75,['{\bf Buck[0] ===>}'],'TexMode','on','horizontalAlignment', 'center')
      | % end
      | 
      | 
      | 
      | port_label('input',1,sprintf('Electrical \nIn'))
      | port_label('input',2,sprintf('Modulation'))
      | % port_label('input',3,'Operating Mode')
      | port_label('output',1,sprintf('Electrical \nOut'))
      | port_label('output',2,sprintf('Cooling \nOut'))
  Inverter_v1 : Subsystem  Commented=on  mask{R1=.01, R2=.01, R3=.01, Cp=60, T_initial=25}
      mask prompts: R1 "Input Voltage Loss Resistance [Ohm]"; R2 "Input Current Loss Resistance [Ohm]"; R3 "Output Voltage Loss Resistance [Ohm]"; Cp "Heat Capacity [J/K]"; T_initial "Initial Temperature [C]"
      mask DialogControl ParameterTabVar0 Prompt: Model Parameters
      mask DialogControl ParameterTabVar01 Prompt: Cooling
      mask DialogControl ParameterTabVar012 Prompt: System
      mask Display:
      | image(imread('inverter.bmp'));
      | text(0.5,0.95,['{\bf Inverter}'],'TexMode','on','horizontalAlignment', 'center')
      | text(0.5,0.075,['{\bf ----(V)}'],'TexMode','on','horizontalAlignment', 'center')
      | 
      | 
      | % switch dir
      | %     case '===>'
      | %         text(0.5,0.85,['{\bf Boost[1] ===>}'],'TexMode','on','horizontalAlignment', 'center')
      | %         text(0.5,0.75,['{\bf Buck[0] <===}'],'TexMode','on','horizontalAlignment', 'center')
      | %     case '<==='
      | %         text(0.5,0.85,['{\bf Boost[1] <===}'],'TexMode','on','horizontalAlignment', 'center')
      | %         text(0.5,0.75,['{\bf Buck[0] ===>}'],'TexMode','on','horizontalAlignment', 'center')
      | % end
      | 
      | 
      | 
      | port_label('input',1,sprintf('Electrical \nIn'))
      | port_label('input',2,sprintf('Duty \nCycle'))
      | % port_label('input',3,'Operating Mode')
      | port_label('output',1,sprintf('Electrical \nOut'))
      | port_label('output',2,sprintf('Cooling \nOut'))
  Motor : Subsystem  AncestorBlock=DAEMOT_Lib_Copy/Dyn Electrical Comp/Motor  mask{m_type=AC, R=0.013461960749493, Kv=0.009688163543703, c=0.000234355495215172, b=1.89435163576232e-05, L=1.252192537082724e-05, J=1.09*10^-4, I_initial=1, w_initial=1, Cp=60, T_initial=25}
      mask prompts: m_type "Motor Type"; R "Armature Resistance [Ohm]"; Kv "Motor Constant [Nm/A] or [V-s/rad]"; c "Static Friction Coefficient [Nm]"; b "Viscous Friction Coefficient [N*m*s/rad]"; L "Armature Inductance [H]"; J "Shaft Inertia [kg*m^2]"; I_initial "Initial Total Current [A]"; w_initial "Initial Speed [rad/s]"; Cp "Motor Heat Capacity [J/K]"; T_initial "Initial Temperature [C]"
      settings: CopyFcn=|
      | h      = get_param(gcb,'handle');   % Get block handle
      | blk    = gcb;
      | 
      | set_param(blk, 'LinkStatus', 'inactive')
      | clear h
      | clear blk
      mask TypeOptions m_type: DC | AC
      mask DialogControl ParameterTabVar0 Prompt: Motor Parameters
      mask DialogControl ParameterTabVar01 Prompt: Cooling
      mask DialogControl ParameterTabVar012 Prompt: System
      mask Display:
      | image(imread('motor.bmp'));
      | T = get_param(gcb,'m_type');
      | if strcmp(T,'DC')
      |     text(0.5,0.95,['{\bf DC Motor}'],'TexMode','on','horizontalAlignment', 'center')
      | else
      |     text(0.5,0.95,['{\bf AC Motor}'],'TexMode','on','horizontalAlignment', 'center')
      | end
      | text(0.5,0.075,['{\bf ---- (end)}'],'TexMode','on','horizontalAlignment', 'center')
      | text(0.5,0.175,['{\bf (start) ----}'],'TexMode','on','horizontalAlignment', 'center')
      | 
      | port_label('input',1,sprintf('Electrical \nIn'))
      | port_label('output',1,sprintf('Mechanical \nOut'))
      | port_label('output',2,sprintf('Cooling \nOut'))
  MotorNoShaft : Subsystem  Commented=on  AncestorBlock=DAEMOT_Lib_Copy/Dyn Electrical Comp/MotorNoShaft  mask{m_type=AC, R=29e-3, Kv=.1238, c=.001, b=1e-5, L=49e-6, I_initial=1, Cp=60, T_initial=25}
      mask prompts: m_type "Motor Type"; R "Armature Resistance [Ohm]"; Kv "Motor Constant [Nm/A] or [V-s/rad]"; c "Static Friction Coefficient [Nm]"; b "Viscous Friction Coefficient [N*m*s/rad]"; L "Armature Inductance [H]"; I_initial "Initial Total Current [A]"; Cp "Motor Heat Capacity [J/K]"; T_initial "Initial Temperature [C]"
      settings: CopyFcn=|
      | h      = get_param(gcb,'handle');   % Get block handle
      | blk    = gcb;
      | 
      | set_param(blk, 'LinkStatus', 'inactive')
      | clear h
      | clear blk
      mask TypeOptions m_type: DC | AC
      mask DialogControl DescTextVar Prompt: For AC machines, parameters are defined using the Power-Invariant Park Transform.
      mask DialogControl ParameterTabVar0 Prompt: Motor Parameters
      mask DialogControl ParameterTabVar01 Prompt: Cooling
      mask DialogControl ParameterTabVar012 Prompt: System
      mask Display:
      | image(imread('motor.bmp'));
      | T = get_param(gcb,'m_type');
      | if strcmp(T,'DC')
      |     text(0.5,0.95,['{\bf DC Motor}'],'TexMode','on','horizontalAlignment', 'center')
      | else
      |     text(0.5,0.95,['{\bf AC Motor}'],'TexMode','on','horizontalAlignment', 'center')
      | end
      | text(0.5,0.075,['{\bf ---- (end)}'],'TexMode','on','horizontalAlignment', 'center')
      | text(0.5,0.175,['{\bf (start) (\tau)}'],'TexMode','on','horizontalAlignment', 'center')
      | 
      | port_label('input',1,sprintf('Electrical \nIn'))
      | port_label('output',1,sprintf('Mechanical \nOut'))
      | port_label('output',2,sprintf('Cooling \nOut'))
  Resistor : Subsystem  mask{r_type=Current, Cp=60, T_initial=25}
      mask prompts: r_type "Resistor Type"; Cp "Heat Capacity [J/K]"; T_initial "Initial Temperature [C]"
      mask init:
      | h      = get_param(gcb,'handle');   % Get block handle
      | blk    = gcb;
      | hblock = get(h);     % Parse out handles structure
      | 
      | if r_type == 1
      |     set_param([blk,'/From8'],'GotoTag',char('out'));
      |     set_param([blk,'/From10'],'GotoTag',char('in'));
      |     set_param([blk,'/From12'],'GotoTag',char('out'));
      |     set_param([blk,'/From4'],'GotoTag',char('out'));
      |     set_param([blk,'/From3'],'GotoTag',char('in'));
      | else
      |     set_param([blk,'/From8'],'GotoTag',char('in'));
      |     set_param([blk,'/From10'],'GotoTag',char('out'));
      |     set_param([blk,'/From12'],'GotoTag',char('in'));
      |     set_param([blk,'/From4'],'GotoTag',char('in'));
      |     set_param([blk,'/From3'],'GotoTag',char('out'));
      | end
      settings: CopyFcn=|
      | h      = get_param(gcb,'handle');   % Get block handle
      | blk    = gcb;
      | 
      | set_param(blk, 'LinkStatus', 'inactive')
      | clear h
      | clear blk
      mask TypeOptions r_type: Voltage | Current
      mask DialogControl ParameterTabVar0 Prompt: Resistor Parameters
      mask DialogControl ParameterTabVar01 Prompt: Cooling
      mask DialogControl ParameterTabVar012 Prompt: System
      mask Display:
      | image(imread('resistor.bmp'));
      | T = get_param(gcb,'r_type');
      | text(0.5,0.95,['{\bf Resistor}'],'TexMode','on','horizontalAlignment', 'center')
      | if strcmp(T,'Current')
      |     text(0.5,0.075,['{\bf (V)*}'],'TexMode','on','horizontalAlignment', 'center')
      | else
      |     text(0.5,0.075,['{\bf ----}'],'TexMode','on','horizontalAlignment', 'center')
      | end
      | port_label('input',1,sprintf('Electrical \nIn'))
      | port_label('input',2,sprintf('Resistance \n[Ohm]'))
      | port_label('output',1,sprintf('Electrical \nOut'))
      | port_label('output',2,sprintf('Cooling \nOut'))
  Shaft : Subsystem  Commented=on  AncestorBlock=DAEMOT_Lib_Copy/Dyn Electrical Comp/Shaft  mask{J=1.09*10^-4, Num_In=1, Num_Out=1, w_initial=0, meme=off}
      mask prompts: J "Shaft Inertia"; Num_In "Number of Inputs"; Num_Out "Number of Outputs"; w_initial "Initial Speed [rad/s]"; meme "Memify"
      mask init:
      | h      = get_param(gcb,'handle');   % Get block handle
      | blk    = gcb;
      | hblock = get(h);     % Parse out handles structure
      | 
      | %%%%%%%%%%%%%%%%%%%%%%%%%%%%%% Clear Stuff %%%%%%%%%%%%%%%%%%%%%%%%%%%%%%%%
      | %delete any previous inports and bus selectors
      | for i = str2num(hblock.Num_In)+1:hblock.Ports(1)
      |     delete_block([blk,'/In',num2str(i)])
      |     delete_block([blk,'/gb',num2str(i)])
      |     delete_block([blk,'/tm',num2str(i)])
      |     delete_block([blk,'/term',num2str(i)])
      |     delete_block([blk,'/Sink',num2str(i)])
      |     delete_block([blk,'/tin',num2str(i)])
      |     
      |     delete_unconnected_lines(blk)
      | end
      | 
      | for i = str2num(hblock.Num_Out)+1:hblock.Ports(2)
      |     delete_block([blk,'/Out',num2str(i)])
      |     delete_block([blk,'/tf',num2str(i)])
      |     delete_block([blk,'/to',num2str(i)])
      |     delete_block([blk,'/b',num2str(i)])
      |     delete_block([blk,'/Source',num2str(i)])
      |     delete_block([blk,'/tg',num2str(i)])
      |     delete_block([blk,'/oo',num2str(i)])
      |     
      |     delete_unconnected_lines(blk)
      | end
      | %%%%%%%%%%%%%%%%%%%%%%%%%%%%% Clear Stuff %%%%%%%%%%%%%%%%%%%%%%%%%%%%%%%%
      | 
      | %%%%%%%%%%%%%%%%%%%%%%%%%%%%%% Edit Mux inputs %%%%%%%%%%%%%%%%%%%%%%%%%%%%%%%%
      | set_param([blk,'/Mux_In_1'],'Inputs',hblock.Num_In)
      | set_param([blk,'/Mux_In_2'],'Inputs',hblock.Num_Out)
      | % set_param([blk,'/Demux_Out_1'],'Outputs',hblock.Num_In)
      | delete_unconnected_lines(blk)
      | 
      | %%%%%%%%%%%%%%%%%%%%%%%%%%%%%% Edit Mux inputs %%%%%%%%%%%%%%%%%%%%%%%%%%%%%%%%
      | 
      | %%%%%%%%%%%%%%%%%%%%%%%%%%%%%% Create and Place Inputs %%%%%%%%%%%%%%%%%%%%%%%%%%%%%%%%
      | % generate inports, bus selectors, and route lines to each vector concat
      | for i = hblock.Ports(1)+1:str2num(hblock.Num_In)
      |     
      |     % add blocks (positioning notation [x i*s+y x+l i*s+h+y] x:(horiz. pos.), y:(vert. pos.), s:(spacing), l:(horiz. length), x:(vert. height)
      |     add_block('simulink/Ports & Subsystems/In1',   [blk,'/In',num2str(i)],    'Position',[355 i*80+425 355+30 i*80+13+425]);         % adding inport
      |     add_block([blk,'/gb1'],                        [blk,'/gb',num2str(i)],   'Position',[440 i*80+410 440+5 i*80+38+410]);         % adding inport
      |     add_block('simulink/Signal Routing/Goto',      [blk,'/tm',num2str(i)],    'Position',[500 i*80+450 500+80 i*80+14+450]);         % adding inport
      |     add_block('simulink/Sinks/Terminator',          [blk,'/term',num2str(i)],    'Position',[500 i*80+415 500+20 i*80+14+415]);         % adding inport
      |     add_block('DAEMOT_Lib/Support Functions/Sink',[blk,'/Sink',num2str(i)],'Position',[200 i*30+336 200+65 i*30+28+336]);         % adding inport
      |     add_block('simulink/Signal Routing/From',       [blk,'/tin',num2str(i)],     'Position',[-400 i*20+405 -400+80 i*20+18+405]);         % adding inport
      |     
      |     % set goto and from tags
      |     set_param([blk,'/tm',num2str(i)],'GotoTag',char(horzcat('tau_in',num2str(i))))
      |     set_param([blk,'/tin',num2str(i)],'GotoTag',char(horzcat('tau_in',num2str(i))))
      |     
      |     % set goto and from background colors
      | %    set_param([blk,'/gm',num2str(i)],'BackgroundColor','yellow')
      | %    set_param([blk,'/gt',num2str(i)],'BackgroundColor','yellow')
      | %    %set_param([blk,'/gp',num2str(i)],'BackgroundColor','yellow')
      | %    set_param([blk,'/min',num2str(i)],'BackgroundColor','yellow')
      | %    set_param([blk,'/tin',num2str(i)],'BackgroundColor','yellow')
      | %    set_param([blk,'/pout',num2str(i)],'BackgroundColor','cyan')
      |     
      |     % add lines
      |     add_line(blk,['In',num2str(i),'/1'], ['gb',num2str(i),'/1'],'AutoRouting','on')
      |     add_line(blk,['gb',num2str(i),'/2'],  ['tm',num2str(i),'/1'],'AutoRouting','on')
      |     add_line(blk,['gb',num2str(i),'/1'],  ['term',num2str(i),'/1'],'AutoRouting','on')
      |     add_line(blk,['Demux_Out_1/',num2str(1)],  ['Sink',num2str(i),'/1'],'AutoRouting','on')
      |     add_line(blk,['tin',num2str(i),'/1'],  ['Mux_In_1/',num2str(i)],'AutoRouting','on')
      |     
      | end
      | %%%%%%%%%%%%%%%%%%%%%%%%%%%%%% Create and Place Inputs %%%%%%%%%%%%%%%%%%%%%%%%%%%%%%%%
      | 
      | %%%%%%%%%%%%%%%%%%%%%%%%%%%%%% Create and Place Outputs %%%%%%%%%%%%%%%%%%%%%%%%%%%%%%%%
      | % generate inports, bus selectors, and route lines to each vector concat
      | for i = hblock.Ports(2)+1:str2num(hblock.Num_Out)
      |     
      |     % add blocks
      |     add_block('simulink/Ports & Subsystems/Out1',   [blk,'/Out',num2str(i)],   'Position',[875 i*80+425 875+30 i*80+13+425]);         % adding inport
      |     add_block('simulink/Signal Routing/Bus Creator',[blk,'/b',num2str(i)],     'Position',[825 i*80+410 825+5 i*80+38+410]);         % adding inport
      |     add_block('simulink/Signal Routing/From',       [blk,'/to',num2str(i)],     'Position',[710 i*80+435 710+80 i*80+14+435]);         % adding inport
      |     add_block('simulink/Signal Routing/From',       [blk,'/oo',num2str(i)],     'Position',[710 i*80+415 710+80 i*80+14+415]);         % adding inport
      |     add_block('simulink/Signal Routing/From',       [blk,'/tf',num2str(i)],     'Position',[935 i*20+410 935+80 i*20+18+410]);         % adding inport
      |     add_block('DAEMOT_Lib/Support Functions/Source',[blk,'/Source',num2str(i)],'Position',[1400 i*30+420 1400+65 i*30+28+420]);         % adding inport
      |     add_block('simulink/Signal Routing/Goto',       [blk,'/tg',num2str(i)],     'Position',[1550 i*30+430 1550+80 i*30+14+430]);         % adding inport
      |     
      |     % set goto and from tags
      |     set_param([blk,'/tf',num2str(i)],'GotoTag',char(horzcat('tau_out',num2str(i))))
      |     set_param([blk,'/to',num2str(i)],'GotoTag',char(horzcat('tau_out',num2str(i))))
      |     set_param([blk,'/oo',num2str(i)],'GotoTag',char(horzcat('omega')))
      |     set_param([blk,'/tg',num2str(i)],'GotoTag',char(horzcat('tau_out',num2str(i))))
      |     set_param([blk,'/b',num2str(i)],'Inputs','2')
      |     
      | %     % set goto and from background colors
      | %     set_param([blk,'/t',num2str(i)],'BackgroundColor','cyan')
      | %     set_param([blk,'/m',num2str(i)],'BackgroundColor','cyan')
      | %     set_param([blk,'/p',num2str(i)],'BackgroundColor','cyan')
      | %     set_param([blk,'/g',num2str(i)],'BackgroundColor','cyan')
      | %     set_param([blk,'/mout',num2str(i)],'BackgroundColor','cyan')
      | %     %set_param([blk,'/tout',num2str(i)],'BackgroundColor','cyan')
      | 
      |     add_line(blk,['oo',num2str(i),'/1'],['b',num2str(i),'/1'],'AutoRouting','on')
      |     p = get_param([blk,'/oo',num2str(i)],'PortHandles');
      |     l = get_param(p.Outport,'Line');
      |     set_param(l,'Name','aspeed')
      |     
      |     add_line(blk,['to',num2str(i),'/1'],['b',num2str(i),'/2'],'AutoRouting','on')
      |     p = get_param([blk,'/to',num2str(i)],'PortHandles');
      |     l = get_param(p.Outport,'Line');
      |     set_param(l,'Name','torque')
      |      
      |     add_line(blk,['b',num2str(i),'/1'],['Out',num2str(i),'/1'],'AutoRouting','on')
      |     add_line(blk,['Source',num2str(i),'/1'],['tg',num2str(i),'/1'],'AutoRouting','on')
      |     add_line(blk,['tf',num2str(i),'/1'],  ['Mux_In_2/',num2str(i)],'AutoRouting','on')
      |     
      | 
      | 
      | end
      | %%%%%%%%%%%%%%%%%%%%%%%%%%%%%% Create and Place Outputs %%%%%%%%%%%%%%%%%%%%%%%%%%%%%%%%
      | 
      | try
      |     set_param([blk,'/Selector1'],'InputPortWidth',num2str(hblock.Num_In))
      |     
      |     selector_str = '[1 ';
      |     for i = 2:str2num(hblock.Num_In)
      |         selector_str = [selector_str,num2str(i),' '];
      |     end
      |     selector_str = [selector_str,']'];
      |     set_param([blk,'/Selector1'],'IndexParamArray',{selector_str})%num2cell(1:hblock.Num_In))
      | catch
      |     selector_str = '[1 ';
      |     for i = 2:str2num(hblock.Num_In)
      |         selector_str = [selector_str,num2str(i),' '];
      |     end
      |     selector_str = [selector_str,']'];
      |     set_param([blk,'/Selector1'],'IndexParamArray',{selector_str})%num2cell(1:hblock.Num_In))
      |     
      |     set_param([blk,'/Selector1'],'InputPortWidth',num2str(hblock.Num_In))
      | end 
      |     
      | try
      |     set_param([blk,'/Selector2'],'InputPortWidth',num2str(hblock.Num_Out))
      |     
      |     selector_str = '[1 ';
      |     for i = 2:str2num(hblock.Num_Out)
      |         selector_str = [selector_str,num2str(i),' '];
      |     end
      |     selector_str = [selector_str,']'];
      |     set_param([blk,'/Selector2'],'IndexParamArray',{selector_str})%num2cell(1:hblock.Num_Out))
      | catch
      |     selector_str = '[1 ';
      |     for i = 2:str2num(hblock.Num_Out)
      |         selector_str = [selector_str,num2str(i),' '];
      |     end
      |     selector_str = [selector_str,']'];
      |     set_param([blk,'/Selector2'],'IndexParamArray',{selector_str})%num2cell(1:hblock.Num_Out))
      |     
      |     set_param([blk,'/Selector2'],'InputPortWidth',num2str(hblock.Num_Out))
      | end 
      | 
      |     clear h blk hblock
      settings: CopyFcn=|
      | h      = get_param(gcb,'handle');   % Get block handle
      | blk    = gcb;
      | 
      | set_param(blk, 'LinkStatus', 'inactive')
      | clear h
      | clear blk
      mask DialogControl ParameterTabVar0 Prompt: Bus Parameters
      mask DialogControl ParameterTabVar01 Prompt: System
      mask Display:
      | meme = get_param(gcb,'meme');
      | if strcmp(meme,'on')
      |     image(imread('ShaftMeme.bmp'));
      | else
      |     image(imread('Shaft.bmp'));
      | end
      | text(0.5,0.95,['{\bf Shaft}'],'TexMode','on','horizontalAlignment', 'center')
      | text(0.5,0.075,['{\bf ----}'],'TexMode','on','horizontalAlignment', 'center')
      | 
      | In = get_param(gcb,'Num_In');
      | Out = get_param(gcb,'Num_Out');
      | 
      | for i = 1:str2num(In)
      |     port_label('input',i,sprintf(['Mech. \nIn ',num2str(i)]))
      | end
      | 
      | for i = 1:str2num(Out)
      |     port_label('output',i,sprintf(['Mech. \nOut ',num2str(i)]))
      | end
  Speed Source : Subsystem  Commented=on  mask(Flow Source (Speed)){M_ext=on, M=0, T_ext=on, T=0, P_ext=on, P=0}
      mask prompts: M_ext "Mass flow rate time varying?"; M "Mass flow rate (kg/s)"; T_ext "Temperature time varying?"; T "Temperature (C)"; P_ext "Pressure time varying?"; P "Pressure (kPa)"
      mask help: Used to create an flow source.
      mask Callback M_ext:
      | en = get_param(gcb,'MaskVisibilities');
      | h      = get_param(gcb,'handle');   % Get block handle
      | blk    = gcb;
      | hblock = get(h);     % Parse out handles structure
      | 
      | switch get_param(gcb,'M_ext')
      |     case 'on'
      |         en{2} = 'off';
      |         %add_block('simulink/Ports & Subsystems/In1',   [blk,'/In1'],'Position',[130    -7   160     7]);         % adding inport
      | 
      |     case 'off'
      |         en{2} = 'on';
      |         %delete_block([blk,'/In1'])
      | 
      | end
      | set_param(gcb,'MaskVisibilities',en);
      mask Callback T_ext:
      | en = get_param(gcb,'MaskVisibilities');
      | 
      | switch get_param(gcb,'T_ext')
      |     case 'on'
      |         en{4} = 'off';
      |     case 'off'
      |         en{4} = 'on';
      | end
      | set_param(gcb,'MaskVisibilities',en);
      mask Callback P_ext:
      | en = get_param(gcb,'MaskVisibilities');
      | 
      | switch get_param(gcb,'P_ext')
      |     case 'on'
      |         en{6} = 'off';
      |     case 'off'
      |         en{6} = 'on';
      | end
      | set_param(gcb,'MaskVisibilities',en);
      mask Display:
      | text(0.5,0.95,['{\bf Flow Source}'],'TexMode','on','horizontalAlignment', 'center')
      | text(0.5,0.1,['{(start) (----)}'],'TexMode','on','horizontalAlignment', 'center')
      | 
      | %port_label('input',1,'Source Torque [Nm]')
      | port_label('input',1,sprintf('Source \nSpeed [rad/s]'))
      | 
      | port_label('output',1,'Source')
  Thermal Sink : Subsystem  Commented=on  mask(Effort Sink (Torque)){M_ext=on, M=0, T_ext=on, T=0, P_ext=on, P=0}
      mask prompts: M_ext "Mass flow rate time varying?"; M "Mass flow rate (kg/s)"; T_ext "Temperature time varying?"; T "Temperature (C)"; P_ext "Pressure time varying?"; P "Pressure (kPa)"
      mask help: Used to create a effot sink.
      mask Callback M_ext:
      | en = get_param(gcb,'MaskVisibilities');
      | h      = get_param(gcb,'handle');   % Get block handle
      | blk    = gcb;
      | hblock = get(h);     % Parse out handles structure
      | 
      | switch get_param(gcb,'M_ext')
      |     case 'on'
      |         en{2} = 'off';
      |         %add_block('simulink/Ports & Subsystems/In1',   [blk,'/In1'],'Position',[130    -7   160     7]);         % adding inport
      | 
      |     case 'off'
      |         en{2} = 'on';
      |         %delete_block([blk,'/In1'])
      | 
      | end
      | set_param(gcb,'MaskVisibilities',en);
      mask Callback T_ext:
      | en = get_param(gcb,'MaskVisibilities');
      | 
      | switch get_param(gcb,'T_ext')
      |     case 'on'
      |         en{4} = 'off';
      |     case 'off'
      |         en{4} = 'on';
      | end
      | set_param(gcb,'MaskVisibilities',en);
      mask Callback P_ext:
      | en = get_param(gcb,'MaskVisibilities');
      | 
      | switch get_param(gcb,'P_ext')
      |     case 'on'
      |         en{6} = 'off';
      |     case 'off'
      |         en{6} = 'on';
      | end
      | set_param(gcb,'MaskVisibilities',en);
      mask Display:
      | text(0.5,0.95,['{\bf Effort Sink}'],'TexMode','on','horizontalAlignment', 'center')
      | text(0.5,0.1,['{(T)(end)}'],'TexMode','on','horizontalAlignment', 'center')
      | 
      | port_label('input',1,'Sink')
      | port_label('input',2,'Sink Temperature [C]')
  Thermal Source : Subsystem  Commented=on  mask(Cooling Source){M_ext=on, M=0, T_ext=on, T=0, P_ext=on, P=0}
      mask prompts: M_ext "Mass flow rate time varying?"; M "Mass flow rate (kg/s)"; T_ext "Temperature time varying?"; T "Temperature (C)"; P_ext "Pressure time varying?"; P "Pressure (kPa)"
      mask help: Used to create an cooling source.
      mask Callback M_ext:
      | en = get_param(gcb,'MaskVisibilities');
      | h      = get_param(gcb,'handle');   % Get block handle
      | blk    = gcb;
      | hblock = get(h);     % Parse out handles structure
      | 
      | switch get_param(gcb,'M_ext')
      |     case 'on'
      |         en{2} = 'off';
      |         %add_block('simulink/Ports & Subsystems/In1',   [blk,'/In1'],'Position',[130    -7   160     7]);         % adding inport
      | 
      |     case 'off'
      |         en{2} = 'on';
      |         %delete_block([blk,'/In1'])
      | 
      | end
      | set_param(gcb,'MaskVisibilities',en);
      mask Callback T_ext:
      | en = get_param(gcb,'MaskVisibilities');
      | 
      | switch get_param(gcb,'T_ext')
      |     case 'on'
      |         en{4} = 'off';
      |     case 'off'
      |         en{4} = 'on';
      | end
      | set_param(gcb,'MaskVisibilities',en);
      mask Callback P_ext:
      | en = get_param(gcb,'MaskVisibilities');
      | 
      | switch get_param(gcb,'P_ext')
      |     case 'on'
      |         en{6} = 'off';
      |     case 'off'
      |         en{6} = 'on';
      | end
      | set_param(gcb,'MaskVisibilities',en);
      mask Display:
      | text(0.5,0.95,['{\bf Effort Source}'],'TexMode','on','horizontalAlignment', 'center')
      | text(0.5,0.1,['{(start)(T)}'],'TexMode','on','horizontalAlignment', 'center')
      | 
      | port_label('input',1,sprintf('Source \nTemperature [C]')  )
      | 
      | port_label('output',1,'Source')
  Torque Sink : Subsystem  Commented=on  mask(Effort Sink (Torque)){M_ext=on, M=0, T_ext=on, T=0, P_ext=on, P=0}
      mask prompts: M_ext "Mass flow rate time varying?"; M "Mass flow rate (kg/s)"; T_ext "Temperature time varying?"; T "Temperature (C)"; P_ext "Pressure time varying?"; P "Pressure (kPa)"
      mask help: Used to create a effot sink.
      mask Callback M_ext:
      | en = get_param(gcb,'MaskVisibilities');
      | h      = get_param(gcb,'handle');   % Get block handle
      | blk    = gcb;
      | hblock = get(h);     % Parse out handles structure
      | 
      | switch get_param(gcb,'M_ext')
      |     case 'on'
      |         en{2} = 'off';
      |         %add_block('simulink/Ports & Subsystems/In1',   [blk,'/In1'],'Position',[130    -7   160     7]);         % adding inport
      | 
      |     case 'off'
      |         en{2} = 'on';
      |         %delete_block([blk,'/In1'])
      | 
      | end
      | set_param(gcb,'MaskVisibilities',en);
      mask Callback T_ext:
      | en = get_param(gcb,'MaskVisibilities');
      | 
      | switch get_param(gcb,'T_ext')
      |     case 'on'
      |         en{4} = 'off';
      |     case 'off'
      |         en{4} = 'on';
      | end
      | set_param(gcb,'MaskVisibilities',en);
      mask Callback P_ext:
      | en = get_param(gcb,'MaskVisibilities');
      | 
      | switch get_param(gcb,'P_ext')
      |     case 'on'
      |         en{6} = 'off';
      |     case 'off'
      |         en{6} = 'on';
      | end
      | set_param(gcb,'MaskVisibilities',en);
      mask Display:
      | text(0.5,0.95,['{\bf Effort Sink}'],'TexMode','on','horizontalAlignment', 'center')
      | text(0.5,0.1,['{(T) (end)}'],'TexMode','on','horizontalAlignment', 'center')
      | 
      | port_label('input',1,'Sink')
      | port_label('input',2,'Sink Torque [Nm]')
  UAV : Subsystem  Commented=on  mask{rho=1.225, d=.8636, b=2, m=69.5*.4536, v_initial=25}
      mask prompts: rho "Air Density [kg/m^3]"; d "Propeller Diameter [m]"; b "Viscous Friction [kg/s]"; m "Vehicle Mass [kg]"; v_initial "Initial Vehicle Speed [m/s]"
      mask init:
      | load('PropellerProp.mat')
      mask DialogControl ParameterTabVar0 Prompt: Capacitor Parameters
      mask DialogControl ParameterTabVar012 Prompt: System
      mask Display:
      | image(imread('UAV.bmp'));
      | text(0.5,0.95,['{\bf UAV}'],'TexMode','on','horizontalAlignment', 'center')
      | text(0.5,0.075,['{\bf (T)  (end)}'],'TexMode','on','horizontalAlignment', 'center')
      | 
      | port_label('input',1,sprintf('Mechanical \nIn'))
  Ultracapacitor : Subsystem  mask(Ultracapacitor){R_cond=1, C_c=34.5, C_s=2, Ns=1, Np=1, UC_ID=Nesscap 100F 2.7V, T_c_0=25, T_s_0=25, V_0=2.3}
      mask prompts: R_cond "Conduction Resistance (K/W)"; C_c "Core Thermal Capacity (J/K)"; C_s "Surface Thermal Capacity (J/K)"; Ns "Number of cells in series"; Np "Number of cells in parallel"; UC_ID "Ultracapacitor Type"; T_c_0 "Initial Core Temperature (C)"; T_s_0 "Initial Surface Temperature (C)"; V_0 "Initial Voltage (V)"
      mask help: Models an ultracapacitor.
      mask init:
      | load('UC_props.mat');
      | 
      | if strcmp(UC_ID,'Nesscap 100F 2.7V')
      |     UC_info = UC_props.NC100F_27V;
      | end
      | 
      | R_i = UC_info.R_i;
      | C_i0 = UC_info.C_i0;
      | C_i1 = UC_info.C_i1;
      | R_d = UC_info.R_d;
      | C_d = UC_info.C_d;
      | R_l = UC_info.R_l;
      | C_l = UC_info.C_l;
      | R_leak = UC_info.R_leak;
      | 
      | % R_i = UC_params(1);
      | % C_i0 = UC_params(2);
      | % C_i1 = UC_params(3);
      | % R_d = UC_params(4);
      | % C_d = UC_params(5);
      | % R_l = UC_params(6);
      | % C_l = UC_params(7);
      | % R_leak = UC_params(8);
      mask TypeOptions UC_ID: Nesscap 100F 2.7V
      mask DialogControl Container14 Prompt: Cell Parameters
      mask DialogControl Container12 Prompt: Initial Conditions
      mask Display:
      | image(imread('ultracapacitor.png'))
      | 
      | N = get_param(gcb,'Np');
      | M = get_param(gcb,'Ns');
      | 
      | text(.5,.92,[M '{\bfS}' N '{\bfP Ultracapacitor}'],'TexMode','on','horizontalAlignment', 'center')
      | 
      | 
      | port_label('input',1,sprintf('Electrical \nIn'))
      | 
      | port_label('output',1,sprintf('Electrical \nOut'))
      | port_label('output',2,sprintf('Cooling \nOut'))
  Voltage Bus : Subsystem  mask(Bus){Num_Out=2}
      mask prompts: Num_Out "Number of Outputs"
      mask help: This is a bus.
      mask init:
      | h      = get_param(gcb,'handle');   % Get block handle
      | blk    = gcb;
      | hblock = get(h);     % Parse out handles structure
      | 
      | %%%%%%%%%%%%%%%%%%%%%%%%%%%%%% Clear Stuff %%%%%%%%%%%%%%%%%%%%%%%%%%%%%%%%
      | % delete any previous inports and bus selectors
      | for i = str2num(hblock.Num_Out)+1:hblock.Ports(2)
      |     delete_block([blk,'/Out',num2str(i)])
      |     delete_block([blk,'/if',num2str(i)])
      |     delete_block([blk,'/io',num2str(i)])
      |     delete_block([blk,'/vo',num2str(i)])
      |     delete_block([blk,'/vot',num2str(i)])
      |     delete_block([blk,'/b',num2str(i)])
      |     delete_block([blk,'/Source',num2str(i)])
      |     delete_block([blk,'/ig',num2str(i)])
      |     delete_block([blk,'/ios',num2str(i)])
      |     delete_block([blk,'/vos',num2str(i)])
      |     
      |     delete_unconnected_lines(blk)
      | end
      | %%%%%%%%%%%%%%%%%%%%%%%%%%%%%% Clear Stuff %%%%%%%%%%%%%%%%%%%%%%%%%%%%%%%%
      | 
      | %%%%%%%%%%%%%%%%%%%%%%%%%%%%%% Edit Mux inputs %%%%%%%%%%%%%%%%%%%%%%%%%%%%%%%%
      | 
      | set_param([blk,'/Mux_In_1'],'Inputs',hblock.Num_Out)
      | set_param([blk,'/Demux_Out_1'],'Outputs',hblock.Num_Out)
      | set_param([blk,'/Bus_Sink_1'],'Inputs',num2str(str2num(hblock.Num_Out)*2))
      | 
      | %%%%%%%%%%%%%%%%%%%%%%%%%%%%%% Edit Mux inputs %%%%%%%%%%%%%%%%%%%%%%%%%%%%%%%%
      | 
      | %%%%%%%%%%%%%%%%%%%%%%%%%%%%%% Creat and Place Outputs %%%%%%%%%%%%%%%%%%%%%%%%%%%%%%%%
      | % generate inports, bus selectors, and route lines to each vector concat
      | for i = hblock.Ports(2)+1:str2num(hblock.Num_Out)
      |     
      |     % add blocks
      |     add_block('simulink/Ports & Subsystems/Out1',   [blk,'/Out',num2str(i)],   'Position',[30 i*80-25-180 60 i*80-12-180]);         % adding inport
      |     add_block('simulink/Signal Routing/From',       [blk,'/io',num2str(i)],     'Position',[-150 i*80-220 -70 i*80-202]);         % adding inport
      |     add_block('simulink/Signal Routing/From',       [blk,'/vo',num2str(i)],     'Position',[-150 i*80-20-180 -70 i*80-2-180]);         % adding inport
      |     add_block('simulink/Signal Routing/Goto',       [blk,'/vot',num2str(i)],     'Position',[1090 i*20-20-250 1170 i*20-2-250]);         % adding inport
      |     add_block('simulink/Signal Routing/From',       [blk,'/if',num2str(i)],     'Position',[25 i*20-20-400 105 i*20-2-400]);         % adding inport
      |     add_block('simulink/Signal Routing/Bus Creator',[blk,'/b',num2str(i)],     'Position',[5 i*80-20+20-218 10 i*80-2+20-198]);         % adding inport
      |     add_block('DAEMOT_Lib/Support Functions/Source',[blk,'/Source',num2str(i)],'Position',[95 i*80-214 160 i*80-186]);         % adding inport
      |     add_block('simulink/Signal Routing/Goto',       [blk,'/ig',num2str(i)],     'Position',[205 i*80-209 285 i*80-191]);         % adding inport
      |     add_block('simulink/Signal Routing/From',       [blk,'/ios',num2str(i)],     'Position',[1000 i*80-20-180 1080 i*80-2-180]);         % adding inport
      |     add_block('simulink/Signal Routing/From',       [blk,'/vos',num2str(i)],     'Position',[1000 i*80-220 1080 i*80-202]);         % adding inport
      |     
      |     % set goto and from tags
      |     set_param([blk,'/if',num2str(i)],'GotoTag',char(horzcat('I_out',num2str(i))))
      |     set_param([blk,'/io',num2str(i)],'GotoTag',char(horzcat('I_out',num2str(i))))
      |     set_param([blk,'/vo',num2str(i)],'GotoTag',char(horzcat('V_out',num2str(i))))
      |     set_param([blk,'/vot',num2str(i)],'GotoTag',char(horzcat('V_out',num2str(i))))
      |     set_param([blk,'/ig',num2str(i)],'GotoTag',char(horzcat('I_out',num2str(i))))
      |     set_param([blk,'/ios',num2str(i)],'GotoTag',char(horzcat('I_out',num2str(i))))
      |     set_param([blk,'/vos',num2str(i)],'GotoTag',char(horzcat('V_out',num2str(i))))    
      |     set_param([blk,'/b',num2str(i)],'Inputs','2')
      |     
      | %     % set goto and from background colors
      | %     set_param([blk,'/t',num2str(i)],'BackgroundColor','cyan')
      | %     set_param([blk,'/m',num2str(i)],'BackgroundColor','cyan')
      | %     set_param([blk,'/p',num2str(i)],'BackgroundColor','cyan')
      | %     set_param([blk,'/g',num2str(i)],'BackgroundColor','cyan')
      | %     set_param([blk,'/mout',num2str(i)],'BackgroundColor','cyan')
      | %     %set_param([blk,'/tout',num2str(i)],'BackgroundColor','cyan')
      |     
      |     % add lines
      |     add_line(blk,['io',num2str(i),'/1'],['b',num2str(i),'/1'],'AutoRouting','on')
      |     p = get_param([blk,'/io',num2str(i)],'PortHandles');
      |     l = get_param(p.Outport,'Line');
      |     set_param(l,'Name','current')
      |     
      |     add_line(blk,['vo',num2str(i),'/1'],['b',num2str(i),'/2'],'AutoRouting','on')
      |     p = get_param([blk,'/vo',num2str(i)],'PortHandles');
      |     l = get_param(p.Outport,'Line');
      |     set_param(l,'Name','voltage')
      |     
      |     % add lines           
      |     add_line(blk,['vos',num2str(i),'/1'],['Bus_Sink_1/',num2str(2*i-1)],'AutoRouting','on')
      |     p = get_param([blk,'/vos',num2str(i)],'PortHandles');
      |     l = get_param(p.Outport,'Line');
      |     set_param(l,'Name',['voltage',num2str(i)])
      |     
      |     add_line(blk,['ios',num2str(i),'/1'],['Bus_Sink_1/',num2str(2*i)],'AutoRouting','on')
      |     p = get_param([blk,'/ios',num2str(i)],'PortHandles');
      |     l = get_param(p.Outport,'Line');
      |     set_param(l,'Name',['current',num2str(i)])
      |      
      |     add_line(blk,['b',num2str(i),'/1'],['Out',num2str(i),'/1'],'AutoRouting','on')
      |     add_line(blk,['Source',num2str(i),'/1'],['ig',num2str(i),'/1'],'AutoRouting','on')
      |     add_line(blk,['if',num2str(i),'/1'],  ['Mux_In_1/',num2str(i)],'AutoRouting','on')
      |     add_line(blk,['Demux_Out_1/',num2str(i)],['vot',num2str(i),'/1'],'AutoRouting','on')
      |     
      | 
      | 
      | end
      | %%%%%%%%%%%%%%%%%%%%%%%%%%%%%% Create and Place Outputs %%%%%%%%%%%%%%%%%%%%%%%%%%%%%%%%
      | 
      | try
      |     set_param([blk,'/Selector1'],'InputPortWidth',num2str(hblock.Num_Out))
      |     
      |     selector_str = '[1 ';
      |     for i = 2:str2num(hblock.Num_Out)
      |         selector_str = [selector_str,num2str(i),' '];
      |     end
      |     selector_str = [selector_str,']'];
      |     set_param([blk,'/Selector1'],'IndexParamArray',{selector_str})%num2cell(1:hblock.Num_Out))
      | catch
      |     selector_str = '[1 ';
      |     for i = 2:str2num(hblock.Num_Out)
      |         selector_str = [selector_str,num2str(i),' '];
      |     end
      |     selector_str = [selector_str,']'];
      |     set_param([blk,'/Selector1'],'IndexParamArray',{selector_str})%num2cell(1:hblock.Num_Out))
      |     
      |     set_param([blk,'/Selector1'],'InputPortWidth',num2str(hblock.Num_Out))
      | end 
      |     
      |     clear h blk hblock
      settings: CopyFcn=|
      | h      = get_param(gcb,'handle');   % Get block handle
      | blk    = gcb;
      | 
      | set_param(blk, 'LinkStatus', 'inactive')
      | clear h
      | clear blk
      mask DialogControl ParameterTabVar0 Prompt: Bus Parameters
      mask DialogControl ParameterTabVar01 Prompt: System
      mask Display:
      | text(0.5,0.95,['{\bf Bus}'],'TexMode','on','horizontalAlignment', 'center')
      | text(0.5,0.075,['{\bf ----(V)}'],'TexMode','on','horizontalAlignment', 'center')
      | 
      | Out = get_param(gcb,'Num_Out');
      | 
      | port_label('input',1,sprintf(['Electrical \nIn ']))
      | port_label('input',2,'u In')
      | 
      | for i = 1:str2num(Out)
      |     port_label('output',i,sprintf(['Electrical \nOut ',num2str(i)]))
      | end
  Voltage Sink : Subsystem  Commented=on  mask(Voltage Sink){M_ext=on, M=0, T_ext=on, T=0, P_ext=on, P=0}
      mask prompts: M_ext "Mass flow rate time varying?"; M "Mass flow rate (kg/s)"; T_ext "Temperature time varying?"; T "Temperature (C)"; P_ext "Pressure time varying?"; P "Pressure (kPa)"
      mask help: Used to create a effort sink.
      mask Callback M_ext:
      | en = get_param(gcb,'MaskVisibilities');
      | h      = get_param(gcb,'handle');   % Get block handle
      | blk    = gcb;
      | hblock = get(h);     % Parse out handles structure
      | 
      | switch get_param(gcb,'M_ext')
      |     case 'on'
      |         en{2} = 'off';
      |         %add_block('simulink/Ports & Subsystems/In1',   [blk,'/In1'],'Position',[130    -7   160     7]);         % adding inport
      | 
      |     case 'off'
      |         en{2} = 'on';
      |         %delete_block([blk,'/In1'])
      | 
      | end
      | set_param(gcb,'MaskVisibilities',en);
      mask Callback T_ext:
      | en = get_param(gcb,'MaskVisibilities');
      | 
      | switch get_param(gcb,'T_ext')
      |     case 'on'
      |         en{4} = 'off';
      |     case 'off'
      |         en{4} = 'on';
      | end
      | set_param(gcb,'MaskVisibilities',en);
      mask Callback P_ext:
      | en = get_param(gcb,'MaskVisibilities');
      | 
      | switch get_param(gcb,'P_ext')
      |     case 'on'
      |         en{6} = 'off';
      |     case 'off'
      |         en{6} = 'on';
      | end
      | set_param(gcb,'MaskVisibilities',en);
      mask Display:
      | text(0.5,0.95,['{\bf Effort Sink}'],'TexMode','on','horizontalAlignment', 'center')
      | text(0.5,0.1,['{(V) (end)}'],'TexMode','on','horizontalAlignment', 'center')
      | 
      | port_label('input',1,'Sink')
      | port_label('input',2,'Sink Voltage [V]')
  Voltage Source : Subsystem  Commented=on  mask(Effort Source (Voltage)){M_ext=on, M=0, T_ext=on, T=0, P_ext=on, P=0}
      mask prompts: M_ext "Mass flow rate time varying?"; M "Mass flow rate (kg/s)"; T_ext "Temperature time varying?"; T "Temperature (C)"; P_ext "Pressure time varying?"; P "Pressure (kPa)"
      mask help: Used to create an effort source.
      mask Callback M_ext:
      | en = get_param(gcb,'MaskVisibilities');
      | h      = get_param(gcb,'handle');   % Get block handle
      | blk    = gcb;
      | hblock = get(h);     % Parse out handles structure
      | 
      | switch get_param(gcb,'M_ext')
      |     case 'on'
      |         en{2} = 'off';
      |         %add_block('simulink/Ports & Subsystems/In1',   [blk,'/In1'],'Position',[130    -7   160     7]);         % adding inport
      | 
      |     case 'off'
      |         en{2} = 'on';
      |         %delete_block([blk,'/In1'])
      | 
      | end
      | set_param(gcb,'MaskVisibilities',en);
      mask Callback T_ext:
      | en = get_param(gcb,'MaskVisibilities');
      | 
      | switch get_param(gcb,'T_ext')
      |     case 'on'
      |         en{4} = 'off';
      |     case 'off'
      |         en{4} = 'on';
      | end
      | set_param(gcb,'MaskVisibilities',en);
      mask Callback P_ext:
      | en = get_param(gcb,'MaskVisibilities');
      | 
      | switch get_param(gcb,'P_ext')
      |     case 'on'
      |         en{6} = 'off';
      |     case 'off'
      |         en{6} = 'on';
      | end
      | set_param(gcb,'MaskVisibilities',en);
      mask Display:
      | text(0.5,0.95,['{\bf Effort Source}'],'TexMode','on','horizontalAlignment', 'center')
      | text(0.5,0.1,['{(start) (V)*}'],'TexMode','on','horizontalAlignment', 'center')
      | 
      | %port_label('input',1,'Source Current [A]')
      | port_label('input',1,sprintf('Source \nVoltage [V]'))
      | 
      | port_label('output',1,'Source')
  wye2del : Subsystem
      settings: CopyFcn=|
      | h      = get_param(gcb,'handle');   % Get block handle
      | blk    = gcb;
      | 
      | set_param(blk, 'LinkStatus', 'inactive')
      | clear h
      | clear blk
      mask DialogControl DescTextVar Prompt: The block converts a wye wound device to a delta wound device.
      mask Display:
      | % image(imread('inverter.bmp'));
      | text(0.5,0.885,['{\bf Y to \Delta}'],'TexMode','on','horizontalAlignment', 'center')
      | text(0.5,0.215,['{\bf ----(V)}'],'TexMode','on','horizontalAlignment', 'center')
      | 
      | 
      | % switch dir
      | %     case '===>'
      | %         text(0.5,0.85,['{\bf Boost[1] ===>}'],'TexMode','on','horizontalAlignment', 'center')
      | %         text(0.5,0.75,['{\bf Buck[0] <===}'],'TexMode','on','horizontalAlignment', 'center')
      | %     case '<==='
      | %         text(0.5,0.85,['{\bf Boost[1] <===}'],'TexMode','on','horizontalAlignment', 'center')
      | %         text(0.5,0.75,['{\bf Buck[0] ===>}'],'TexMode','on','horizontalAlignment', 'center')
      | % end
      | 
      | 
      | 
      | port_label('input',1,sprintf('Electrical \nIn'))
      | % port_label('input',3,'Operating Mode')
      | port_label('output',1,sprintf('Electrical \nOut'))
